simulink model "HornetXII_Challenge"  (R2026a)
settings: Solver=VariableStepAuto  StopTime=300  AbsTol=1e-3  EnableMultiTasking=on
InitFcn:
  | searchHalfSpan = 5;
  | 
  | rng('shuffle');
  | Environment.target.seed = randi(2^31 - 1);
  | 
  | % Use the saved seed to make this particular run reproducible if needed.
  | rng(Environment.target.seed, 'twister');
  | 
  | Environment.target.xy = (2*rand(2,1) - 1) * searchHalfSpan;
  | 
  | Environment.target.pos = [Environment.target.xy;
  |     Environment.seafloordepth - Environment.target.side/2];
values from neighbouring files (symbols this model uses):
  N = size(Vehicle.thrusterori, 2)    [VehicleParameters.m]
undefined symbols (not defined in the file or in its folder): B, pospoints, Spline, timepoints, Vehicle, X, Y, Z
libraries: sm_lib x554, nesl_utility x23, slpidlib x13, matrix_library x4, robotcorelib x2, fl_lib x1, simulink x1
(part 3 of 14)

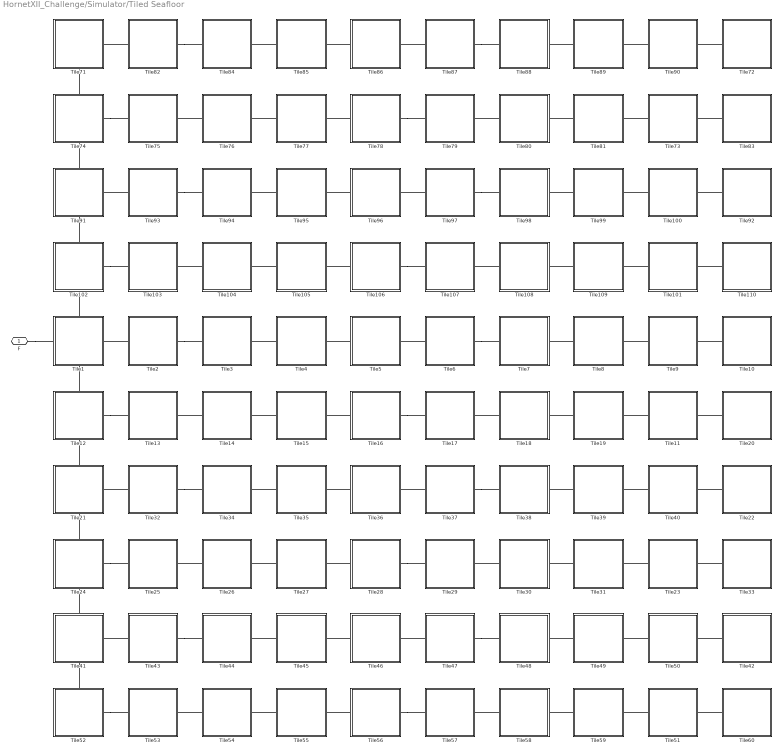
== system HornetXII_Challenge/Simulator/Tiled Seafloor ==
  Tile1 : Subsystem  mask(Square Tile){side=side, thickness=thick, color=color1, opacity=opacity}
      mask prompts: side "Side (m) :"; thickness "Thickness (m) :"; color "Color [RGB] :"; opacity "Opacity (0...1) :"
      mask help: This block creates a flat, single, square tile element. The square tile body is mass-less, so it will not have an effect on the dynamic simulation. This square tile element can be used as a graphic reference by itself, or as part of a composite graphic reference made of an array of interconnected tiles. The square tile is aligned with the XY plane, and the block provides frame connector ports to the middle points on each of the four sides of the body of the square - right (+X), left (-X), top (+Y) and bottom (-Y). All dimensions are in meters.
      settings: PortSchema="{\"entries\":[{\"content\":{\"sides\":[{\"content\":{\"connectorIds\":[\"LConn1\"]},\"type\":\"ConnectorPlacement.EquallySpacedRectSide\",\"uuid\":\"a971723f-ea37-4e9b-910b-501b94fb0ba2\"},{\"content\":{\"connectorIds\":[\"RConn1\"],\"side\":\"RIGHT\"},\"type\":\"ConnectorPlacement.EquallySpacedRectSide\",\"uuid\":\"e50175c1-005c-4b0b-bced-b882197eaab2\"},{\"content\":{\"connectorIds\":[\"LConn2\"],\"side\":\"TOP\"},\"type\":\"ConnectorPlacement.EquallySpacedRectSide\",\"uuid\":\"2a04a964-d53e-47ee-8c79-d53dd599bafe\"},{\"content\":{\"connectorIds\":[\"RConn2\"],\"side\":\"BOTTOM\"},\"type\":\"ConnectorPlacement.EquallySpacedRectSide\",\"uuid\":\"a0066dd6-a193-491c-afbe-bac00dfc3505\"}]},\"type\":\"ConnectorPlacement.EquallySpacedConnector\",\"uuid\":\"c80211c6-bb24-481b-97ca-2752015f3b18\"}],\"packageUris\":[\"http://schema.mathworks.com/mf0/Connector/19700101\"],\"version\":\"1.0\"}"
  Tile10 : Subsystem  mask(Square Tile){side=side, thickness=thick, color=color2, opacity=opacity}
      mask prompts: side "Side (m) :"; thickness "Thickness (m) :"; color "Color [RGB] :"; opacity "Opacity (0...1) :"
      mask help: This block creates a flat, single, square tile element. The square tile body is mass-less, so it will not have an effect on the dynamic simulation. This square tile element can be used as a graphic reference by itself, or as part of a composite graphic reference made of an array of interconnected tiles. The square tile is aligned with the XY plane, and the block provides frame connector ports to the middle points on each of the four sides of the body of the square - right (+X), left (-X), top (+Y) and bottom (-Y). All dimensions are in meters.
      settings: PortSchema="{\"entries\":[{\"content\":{\"sides\":[{\"content\":{\"connectorIds\":[\"LConn1\"]},\"type\":\"ConnectorPlacement.EquallySpacedRectSide\",\"uuid\":\"a971723f-ea37-4e9b-910b-501b94fb0ba2\"},{\"content\":{\"connectorIds\":[\"RConn1\"],\"side\":\"RIGHT\"},\"type\":\"ConnectorPlacement.EquallySpacedRectSide\",\"uuid\":\"e50175c1-005c-4b0b-bced-b882197eaab2\"},{\"content\":{\"connectorIds\":[\"LConn2\"],\"side\":\"TOP\"},\"type\":\"ConnectorPlacement.EquallySpacedRectSide\",\"uuid\":\"2a04a964-d53e-47ee-8c79-d53dd599bafe\"},{\"content\":{\"connectorIds\":[\"RConn2\"],\"side\":\"BOTTOM\"},\"type\":\"ConnectorPlacement.EquallySpacedRectSide\",\"uuid\":\"a0066dd6-a193-491c-afbe-bac00dfc3505\"}]},\"type\":\"ConnectorPlacement.EquallySpacedConnector\",\"uuid\":\"c80211c6-bb24-481b-97ca-2752015f3b18\"}],\"packageUris\":[\"http://schema.mathworks.com/mf0/Connector/19700101\"],\"version\":\"1.0\"}"
  Tile100 : Subsystem  mask(Square Tile){side=side, thickness=thick, color=color1, opacity=opacity}
      mask prompts: side "Side (m) :"; thickness "Thickness (m) :"; color "Color [RGB] :"; opacity "Opacity (0...1) :"
      mask help: This block creates a flat, single, square tile element. The square tile body is mass-less, so it will not have an effect on the dynamic simulation. This square tile element can be used as a graphic reference by itself, or as part of a composite graphic reference made of an array of interconnected tiles. The square tile is aligned with the XY plane, and the block provides frame connector ports to the middle points on each of the four sides of the body of the square - right (+X), left (-X), top (+Y) and bottom (-Y). All dimensions are in meters.
      settings: PortSchema="{\"entries\":[{\"content\":{\"sides\":[{\"content\":{\"connectorIds\":[\"LConn1\"]},\"type\":\"ConnectorPlacement.EquallySpacedRectSide\",\"uuid\":\"a971723f-ea37-4e9b-910b-501b94fb0ba2\"},{\"content\":{\"connectorIds\":[\"RConn1\"],\"side\":\"RIGHT\"},\"type\":\"ConnectorPlacement.EquallySpacedRectSide\",\"uuid\":\"e50175c1-005c-4b0b-bced-b882197eaab2\"},{\"content\":{\"connectorIds\":[\"LConn2\"],\"side\":\"TOP\"},\"type\":\"ConnectorPlacement.EquallySpacedRectSide\",\"uuid\":\"2a04a964-d53e-47ee-8c79-d53dd599bafe\"},{\"content\":{\"connectorIds\":[\"RConn2\"],\"side\":\"BOTTOM\"},\"type\":\"ConnectorPlacement.EquallySpacedRectSide\",\"uuid\":\"a0066dd6-a193-491c-afbe-bac00dfc3505\"}]},\"type\":\"ConnectorPlacement.EquallySpacedConnector\",\"uuid\":\"c80211c6-bb24-481b-97ca-2752015f3b18\"}],\"packageUris\":[\"http://schema.mathworks.com/mf0/Connector/19700101\"],\"version\":\"1.0\"}"
  Tile101 : Subsystem  mask(Square Tile){side=side, thickness=thick, color=color2, opacity=opacity}
      mask prompts: side "Side (m) :"; thickness "Thickness (m) :"; color "Color [RGB] :"; opacity "Opacity (0...1) :"
      mask help: This block creates a flat, single, square tile element. The square tile body is mass-less, so it will not have an effect on the dynamic simulation. This square tile element can be used as a graphic reference by itself, or as part of a composite graphic reference made of an array of interconnected tiles. The square tile is aligned with the XY plane, and the block provides frame connector ports to the middle points on each of the four sides of the body of the square - right (+X), left (-X), top (+Y) and bottom (-Y). All dimensions are in meters.
      settings: PortSchema="{\"entries\":[{\"content\":{\"sides\":[{\"content\":{\"connectorIds\":[\"LConn1\"]},\"type\":\"ConnectorPlacement.EquallySpacedRectSide\",\"uuid\":\"a971723f-ea37-4e9b-910b-501b94fb0ba2\"},{\"content\":{\"connectorIds\":[\"RConn1\"],\"side\":\"RIGHT\"},\"type\":\"ConnectorPlacement.EquallySpacedRectSide\",\"uuid\":\"e50175c1-005c-4b0b-bced-b882197eaab2\"},{\"content\":{\"connectorIds\":[\"LConn2\"],\"side\":\"TOP\"},\"type\":\"ConnectorPlacement.EquallySpacedRectSide\",\"uuid\":\"2a04a964-d53e-47ee-8c79-d53dd599bafe\"},{\"content\":{\"connectorIds\":[\"RConn2\"],\"side\":\"BOTTOM\"},\"type\":\"ConnectorPlacement.EquallySpacedRectSide\",\"uuid\":\"a0066dd6-a193-491c-afbe-bac00dfc3505\"}]},\"type\":\"ConnectorPlacement.EquallySpacedConnector\",\"uuid\":\"c80211c6-bb24-481b-97ca-2752015f3b18\"}],\"packageUris\":[\"http://schema.mathworks.com/mf0/Connector/19700101\"],\"version\":\"1.0\"}"
  Tile102 : Subsystem  mask(Square Tile){side=side, thickness=thick, color=color2, opacity=opacity}
      mask prompts: side "Side (m) :"; thickness "Thickness (m) :"; color "Color [RGB] :"; opacity "Opacity (0...1) :"
      mask help: This block creates a flat, single, square tile element. The square tile body is mass-less, so it will not have an effect on the dynamic simulation. This square tile element can be used as a graphic reference by itself, or as part of a composite graphic reference made of an array of interconnected tiles. The square tile is aligned with the XY plane, and the block provides frame connector ports to the middle points on each of the four sides of the body of the square - right (+X), left (-X), top (+Y) and bottom (-Y). All dimensions are in meters.
      settings: PortSchema="{\"entries\":[{\"content\":{\"sides\":[{\"content\":{\"connectorIds\":[\"LConn1\"]},\"type\":\"ConnectorPlacement.EquallySpacedRectSide\",\"uuid\":\"a971723f-ea37-4e9b-910b-501b94fb0ba2\"},{\"content\":{\"connectorIds\":[\"RConn1\"],\"side\":\"RIGHT\"},\"type\":\"ConnectorPlacement.EquallySpacedRectSide\",\"uuid\":\"e50175c1-005c-4b0b-bced-b882197eaab2\"},{\"content\":{\"connectorIds\":[\"LConn2\"],\"side\":\"TOP\"},\"type\":\"ConnectorPlacement.EquallySpacedRectSide\",\"uuid\":\"2a04a964-d53e-47ee-8c79-d53dd599bafe\"},{\"content\":{\"connectorIds\":[\"RConn2\"],\"side\":\"BOTTOM\"},\"type\":\"ConnectorPlacement.EquallySpacedRectSide\",\"uuid\":\"a0066dd6-a193-491c-afbe-bac00dfc3505\"}]},\"type\":\"ConnectorPlacement.EquallySpacedConnector\",\"uuid\":\"c80211c6-bb24-481b-97ca-2752015f3b18\"}],\"packageUris\":[\"http://schema.mathworks.com/mf0/Connector/19700101\"],\"version\":\"1.0\"}"
  Tile103 : Subsystem  mask(Square Tile){side=side, thickness=thick, color=color1, opacity=opacity}
      mask prompts: side "Side (m) :"; thickness "Thickness (m) :"; color "Color [RGB] :"; opacity "Opacity (0...1) :"
      mask help: This block creates a flat, single, square tile element. The square tile body is mass-less, so it will not have an effect on the dynamic simulation. This square tile element can be used as a graphic reference by itself, or as part of a composite graphic reference made of an array of interconnected tiles. The square tile is aligned with the XY plane, and the block provides frame connector ports to the middle points on each of the four sides of the body of the square - right (+X), left (-X), top (+Y) and bottom (-Y). All dimensions are in meters.
      settings: PortSchema="{\"entries\":[{\"content\":{\"sides\":[{\"content\":{\"connectorIds\":[\"LConn1\"]},\"type\":\"ConnectorPlacement.EquallySpacedRectSide\",\"uuid\":\"a971723f-ea37-4e9b-910b-501b94fb0ba2\"},{\"content\":{\"connectorIds\":[\"RConn1\"],\"side\":\"RIGHT\"},\"type\":\"ConnectorPlacement.EquallySpacedRectSide\",\"uuid\":\"e50175c1-005c-4b0b-bced-b882197eaab2\"},{\"content\":{\"connectorIds\":[\"LConn2\"],\"side\":\"TOP\"},\"type\":\"ConnectorPlacement.EquallySpacedRectSide\",\"uuid\":\"2a04a964-d53e-47ee-8c79-d53dd599bafe\"},{\"content\":{\"connectorIds\":[\"RConn2\"],\"side\":\"BOTTOM\"},\"type\":\"ConnectorPlacement.EquallySpacedRectSide\",\"uuid\":\"a0066dd6-a193-491c-afbe-bac00dfc3505\"}]},\"type\":\"ConnectorPlacement.EquallySpacedConnector\",\"uuid\":\"c80211c6-bb24-481b-97ca-2752015f3b18\"}],\"packageUris\":[\"http://schema.mathworks.com/mf0/Connector/19700101\"],\"version\":\"1.0\"}"
  Tile104 : Subsystem  mask(Square Tile){side=side, thickness=thick, color=color2, opacity=opacity}
      mask prompts: side "Side (m) :"; thickness "Thickness (m) :"; color "Color [RGB] :"; opacity "Opacity (0...1) :"
      mask help: This block creates a flat, single, square tile element. The square tile body is mass-less, so it will not have an effect on the dynamic simulation. This square tile element can be used as a graphic reference by itself, or as part of a composite graphic reference made of an array of interconnected tiles. The square tile is aligned with the XY plane, and the block provides frame connector ports to the middle points on each of the four sides of the body of the square - right (+X), left (-X), top (+Y) and bottom (-Y). All dimensions are in meters.
      settings: PortSchema="{\"entries\":[{\"content\":{\"sides\":[{\"content\":{\"connectorIds\":[\"LConn1\"]},\"type\":\"ConnectorPlacement.EquallySpacedRectSide\",\"uuid\":\"a971723f-ea37-4e9b-910b-501b94fb0ba2\"},{\"content\":{\"connectorIds\":[\"RConn1\"],\"side\":\"RIGHT\"},\"type\":\"ConnectorPlacement.EquallySpacedRectSide\",\"uuid\":\"e50175c1-005c-4b0b-bced-b882197eaab2\"},{\"content\":{\"connectorIds\":[\"LConn2\"],\"side\":\"TOP\"},\"type\":\"ConnectorPlacement.EquallySpacedRectSide\",\"uuid\":\"2a04a964-d53e-47ee-8c79-d53dd599bafe\"},{\"content\":{\"connectorIds\":[\"RConn2\"],\"side\":\"BOTTOM\"},\"type\":\"ConnectorPlacement.EquallySpacedRectSide\",\"uuid\":\"a0066dd6-a193-491c-afbe-bac00dfc3505\"}]},\"type\":\"ConnectorPlacement.EquallySpacedConnector\",\"uuid\":\"c80211c6-bb24-481b-97ca-2752015f3b18\"}],\"packageUris\":[\"http://schema.mathworks.com/mf0/Connector/19700101\"],\"version\":\"1.0\"}"
  Tile105 : Subsystem  mask(Square Tile){side=side, thickness=thick, color=color1, opacity=opacity}
      mask prompts: side "Side (m) :"; thickness "Thickness (m) :"; color "Color [RGB] :"; opacity "Opacity (0...1) :"
      mask help: This block creates a flat, single, square tile element. The square tile body is mass-less, so it will not have an effect on the dynamic simulation. This square tile element can be used as a graphic reference by itself, or as part of a composite graphic reference made of an array of interconnected tiles. The square tile is aligned with the XY plane, and the block provides frame connector ports to the middle points on each of the four sides of the body of the square - right (+X), left (-X), top (+Y) and bottom (-Y). All dimensions are in meters.
      settings: PortSchema="{\"entries\":[{\"content\":{\"sides\":[{\"content\":{\"connectorIds\":[\"LConn1\"]},\"type\":\"ConnectorPlacement.EquallySpacedRectSide\",\"uuid\":\"a971723f-ea37-4e9b-910b-501b94fb0ba2\"},{\"content\":{\"connectorIds\":[\"RConn1\"],\"side\":\"RIGHT\"},\"type\":\"ConnectorPlacement.EquallySpacedRectSide\",\"uuid\":\"e50175c1-005c-4b0b-bced-b882197eaab2\"},{\"content\":{\"connectorIds\":[\"LConn2\"],\"side\":\"TOP\"},\"type\":\"ConnectorPlacement.EquallySpacedRectSide\",\"uuid\":\"2a04a964-d53e-47ee-8c79-d53dd599bafe\"},{\"content\":{\"connectorIds\":[\"RConn2\"],\"side\":\"BOTTOM\"},\"type\":\"ConnectorPlacement.EquallySpacedRectSide\",\"uuid\":\"a0066dd6-a193-491c-afbe-bac00dfc3505\"}]},\"type\":\"ConnectorPlacement.EquallySpacedConnector\",\"uuid\":\"c80211c6-bb24-481b-97ca-2752015f3b18\"}],\"packageUris\":[\"http://schema.mathworks.com/mf0/Connector/19700101\"],\"version\":\"1.0\"}"
  Tile106 : Subsystem  mask(Square Tile){side=side, thickness=thick, color=color2, opacity=opacity}
      mask prompts: side "Side (m) :"; thickness "Thickness (m) :"; color "Color [RGB] :"; opacity "Opacity (0...1) :"
      mask help: This block creates a flat, single, square tile element. The square tile body is mass-less, so it will not have an effect on the dynamic simulation. This square tile element can be used as a graphic reference by itself, or as part of a composite graphic reference made of an array of interconnected tiles. The square tile is aligned with the XY plane, and the block provides frame connector ports to the middle points on each of the four sides of the body of the square - right (+X), left (-X), top (+Y) and bottom (-Y). All dimensions are in meters.
      settings: PortSchema="{\"entries\":[{\"content\":{\"sides\":[{\"content\":{\"connectorIds\":[\"LConn1\"]},\"type\":\"ConnectorPlacement.EquallySpacedRectSide\",\"uuid\":\"a971723f-ea37-4e9b-910b-501b94fb0ba2\"},{\"content\":{\"connectorIds\":[\"RConn1\"],\"side\":\"RIGHT\"},\"type\":\"ConnectorPlacement.EquallySpacedRectSide\",\"uuid\":\"e50175c1-005c-4b0b-bced-b882197eaab2\"},{\"content\":{\"connectorIds\":[\"LConn2\"],\"side\":\"TOP\"},\"type\":\"ConnectorPlacement.EquallySpacedRectSide\",\"uuid\":\"2a04a964-d53e-47ee-8c79-d53dd599bafe\"},{\"content\":{\"connectorIds\":[\"RConn2\"],\"side\":\"BOTTOM\"},\"type\":\"ConnectorPlacement.EquallySpacedRectSide\",\"uuid\":\"a0066dd6-a193-491c-afbe-bac00dfc3505\"}]},\"type\":\"ConnectorPlacement.EquallySpacedConnector\",\"uuid\":\"c80211c6-bb24-481b-97ca-2752015f3b18\"}],\"packageUris\":[\"http://schema.mathworks.com/mf0/Connector/19700101\"],\"version\":\"1.0\"}"
  Tile107 : Subsystem  mask(Square Tile){side=side, thickness=thick, color=color1, opacity=opacity}
      mask prompts: side "Side (m) :"; thickness "Thickness (m) :"; color "Color [RGB] :"; opacity "Opacity (0...1) :"
      mask help: This block creates a flat, single, square tile element. The square tile body is mass-less, so it will not have an effect on the dynamic simulation. This square tile element can be used as a graphic reference by itself, or as part of a composite graphic reference made of an array of interconnected tiles. The square tile is aligned with the XY plane, and the block provides frame connector ports to the middle points on each of the four sides of the body of the square - right (+X), left (-X), top (+Y) and bottom (-Y). All dimensions are in meters.
      settings: PortSchema="{\"entries\":[{\"content\":{\"sides\":[{\"content\":{\"connectorIds\":[\"LConn1\"]},\"type\":\"ConnectorPlacement.EquallySpacedRectSide\",\"uuid\":\"a971723f-ea37-4e9b-910b-501b94fb0ba2\"},{\"content\":{\"connectorIds\":[\"RConn1\"],\"side\":\"RIGHT\"},\"type\":\"ConnectorPlacement.EquallySpacedRectSide\",\"uuid\":\"e50175c1-005c-4b0b-bced-b882197eaab2\"},{\"content\":{\"connectorIds\":[\"LConn2\"],\"side\":\"TOP\"},\"type\":\"ConnectorPlacement.EquallySpacedRectSide\",\"uuid\":\"2a04a964-d53e-47ee-8c79-d53dd599bafe\"},{\"content\":{\"connectorIds\":[\"RConn2\"],\"side\":\"BOTTOM\"},\"type\":\"ConnectorPlacement.EquallySpacedRectSide\",\"uuid\":\"a0066dd6-a193-491c-afbe-bac00dfc3505\"}]},\"type\":\"ConnectorPlacement.EquallySpacedConnector\",\"uuid\":\"c80211c6-bb24-481b-97ca-2752015f3b18\"}],\"packageUris\":[\"http://schema.mathworks.com/mf0/Connector/19700101\"],\"version\":\"1.0\"}"
  Tile108 : Subsystem  mask(Square Tile){side=side, thickness=thick, color=color2, opacity=opacity}
      mask prompts: side "Side (m) :"; thickness "Thickness (m) :"; color "Color [RGB] :"; opacity "Opacity (0...1) :"
      mask help: This block creates a flat, single, square tile element. The square tile body is mass-less, so it will not have an effect on the dynamic simulation. This square tile element can be used as a graphic reference by itself, or as part of a composite graphic reference made of an array of interconnected tiles. The square tile is aligned with the XY plane, and the block provides frame connector ports to the middle points on each of the four sides of the body of the square - right (+X), left (-X), top (+Y) and bottom (-Y). All dimensions are in meters.
      settings: PortSchema="{\"entries\":[{\"content\":{\"sides\":[{\"content\":{\"connectorIds\":[\"LConn1\"]},\"type\":\"ConnectorPlacement.EquallySpacedRectSide\",\"uuid\":\"a971723f-ea37-4e9b-910b-501b94fb0ba2\"},{\"content\":{\"connectorIds\":[\"RConn1\"],\"side\":\"RIGHT\"},\"type\":\"ConnectorPlacement.EquallySpacedRectSide\",\"uuid\":\"e50175c1-005c-4b0b-bced-b882197eaab2\"},{\"content\":{\"connectorIds\":[\"LConn2\"],\"side\":\"TOP\"},\"type\":\"ConnectorPlacement.EquallySpacedRectSide\",\"uuid\":\"2a04a964-d53e-47ee-8c79-d53dd599bafe\"},{\"content\":{\"connectorIds\":[\"RConn2\"],\"side\":\"BOTTOM\"},\"type\":\"ConnectorPlacement.EquallySpacedRectSide\",\"uuid\":\"a0066dd6-a193-491c-afbe-bac00dfc3505\"}]},\"type\":\"ConnectorPlacement.EquallySpacedConnector\",\"uuid\":\"c80211c6-bb24-481b-97ca-2752015f3b18\"}],\"packageUris\":[\"http://schema.mathworks.com/mf0/Connector/19700101\"],\"version\":\"1.0\"}"
  Tile109 : Subsystem  mask(Square Tile){side=side, thickness=thick, color=color1, opacity=opacity}
      mask prompts: side "Side (m) :"; thickness "Thickness (m) :"; color "Color [RGB] :"; opacity "Opacity (0...1) :"
      mask help: This block creates a flat, single, square tile element. The square tile body is mass-less, so it will not have an effect on the dynamic simulation. This square tile element can be used as a graphic reference by itself, or as part of a composite graphic reference made of an array of interconnected tiles. The square tile is aligned with the XY plane, and the block provides frame connector ports to the middle points on each of the four sides of the body of the square - right (+X), left (-X), top (+Y) and bottom (-Y). All dimensions are in meters.
      settings: PortSchema="{\"entries\":[{\"content\":{\"sides\":[{\"content\":{\"connectorIds\":[\"LConn1\"]},\"type\":\"ConnectorPlacement.EquallySpacedRectSide\",\"uuid\":\"a971723f-ea37-4e9b-910b-501b94fb0ba2\"},{\"content\":{\"connectorIds\":[\"RConn1\"],\"side\":\"RIGHT\"},\"type\":\"ConnectorPlacement.EquallySpacedRectSide\",\"uuid\":\"e50175c1-005c-4b0b-bced-b882197eaab2\"},{\"content\":{\"connectorIds\":[\"LConn2\"],\"side\":\"TOP\"},\"type\":\"ConnectorPlacement.EquallySpacedRectSide\",\"uuid\":\"2a04a964-d53e-47ee-8c79-d53dd599bafe\"},{\"content\":{\"connectorIds\":[\"RConn2\"],\"side\":\"BOTTOM\"},\"type\":\"ConnectorPlacement.EquallySpacedRectSide\",\"uuid\":\"a0066dd6-a193-491c-afbe-bac00dfc3505\"}]},\"type\":\"ConnectorPlacement.EquallySpacedConnector\",\"uuid\":\"c80211c6-bb24-481b-97ca-2752015f3b18\"}],\"packageUris\":[\"http://schema.mathworks.com/mf0/Connector/19700101\"],\"version\":\"1.0\"}"
  Tile11 : Subsystem  mask(Square Tile){side=side, thickness=thick, color=color2, opacity=opacity}
      mask prompts: side "Side (m) :"; thickness "Thickness (m) :"; color "Color [RGB] :"; opacity "Opacity (0...1) :"
      mask help: This block creates a flat, single, square tile element. The square tile body is mass-less, so it will not have an effect on the dynamic simulation. This square tile element can be used as a graphic reference by itself, or as part of a composite graphic reference made of an array of interconnected tiles. The square tile is aligned with the XY plane, and the block provides frame connector ports to the middle points on each of the four sides of the body of the square - right (+X), left (-X), top (+Y) and bottom (-Y). All dimensions are in meters.
      settings: PortSchema="{\"entries\":[{\"content\":{\"sides\":[{\"content\":{\"connectorIds\":[\"LConn1\"]},\"type\":\"ConnectorPlacement.EquallySpacedRectSide\",\"uuid\":\"a971723f-ea37-4e9b-910b-501b94fb0ba2\"},{\"content\":{\"connectorIds\":[\"RConn1\"],\"side\":\"RIGHT\"},\"type\":\"ConnectorPlacement.EquallySpacedRectSide\",\"uuid\":\"e50175c1-005c-4b0b-bced-b882197eaab2\"},{\"content\":{\"connectorIds\":[\"LConn2\"],\"side\":\"TOP\"},\"type\":\"ConnectorPlacement.EquallySpacedRectSide\",\"uuid\":\"2a04a964-d53e-47ee-8c79-d53dd599bafe\"},{\"content\":{\"connectorIds\":[\"RConn2\"],\"side\":\"BOTTOM\"},\"type\":\"ConnectorPlacement.EquallySpacedRectSide\",\"uuid\":\"a0066dd6-a193-491c-afbe-bac00dfc3505\"}]},\"type\":\"ConnectorPlacement.EquallySpacedConnector\",\"uuid\":\"c80211c6-bb24-481b-97ca-2752015f3b18\"}],\"packageUris\":[\"http://schema.mathworks.com/mf0/Connector/19700101\"],\"version\":\"1.0\"}"
  Tile110 : Subsystem  mask(Square Tile){side=side, thickness=thick, color=color1, opacity=opacity}
      mask prompts: side "Side (m) :"; thickness "Thickness (m) :"; color "Color [RGB] :"; opacity "Opacity (0...1) :"
      mask help: This block creates a flat, single, square tile element. The square tile body is mass-less, so it will not have an effect on the dynamic simulation. This square tile element can be used as a graphic reference by itself, or as part of a composite graphic reference made of an array of interconnected tiles. The square tile is aligned with the XY plane, and the block provides frame connector ports to the middle points on each of the four sides of the body of the square - right (+X), left (-X), top (+Y) and bottom (-Y). All dimensions are in meters.
      settings: PortSchema="{\"entries\":[{\"content\":{\"sides\":[{\"content\":{\"connectorIds\":[\"LConn1\"]},\"type\":\"ConnectorPlacement.EquallySpacedRectSide\",\"uuid\":\"a971723f-ea37-4e9b-910b-501b94fb0ba2\"},{\"content\":{\"connectorIds\":[\"RConn1\"],\"side\":\"RIGHT\"},\"type\":\"ConnectorPlacement.EquallySpacedRectSide\",\"uuid\":\"e50175c1-005c-4b0b-bced-b882197eaab2\"},{\"content\":{\"connectorIds\":[\"LConn2\"],\"side\":\"TOP\"},\"type\":\"ConnectorPlacement.EquallySpacedRectSide\",\"uuid\":\"2a04a964-d53e-47ee-8c79-d53dd599bafe\"},{\"content\":{\"connectorIds\":[\"RConn2\"],\"side\":\"BOTTOM\"},\"type\":\"ConnectorPlacement.EquallySpacedRectSide\",\"uuid\":\"a0066dd6-a193-491c-afbe-bac00dfc3505\"}]},\"type\":\"ConnectorPlacement.EquallySpacedConnector\",\"uuid\":\"c80211c6-bb24-481b-97ca-2752015f3b18\"}],\"packageUris\":[\"http://schema.mathworks.com/mf0/Connector/19700101\"],\"version\":\"1.0\"}"
  Tile12 : Subsystem  mask(Square Tile){side=side, thickness=thick, color=color2, opacity=opacity}
      mask prompts: side "Side (m) :"; thickness "Thickness (m) :"; color "Color [RGB] :"; opacity "Opacity (0...1) :"
      mask help: This block creates a flat, single, square tile element. The square tile body is mass-less, so it will not have an effect on the dynamic simulation. This square tile element can be used as a graphic reference by itself, or as part of a composite graphic reference made of an array of interconnected tiles. The square tile is aligned with the XY plane, and the block provides frame connector ports to the middle points on each of the four sides of the body of the square - right (+X), left (-X), top (+Y) and bottom (-Y). All dimensions are in meters.
      settings: PortSchema="{\"entries\":[{\"content\":{\"sides\":[{\"content\":{\"connectorIds\":[\"LConn1\"]},\"type\":\"ConnectorPlacement.EquallySpacedRectSide\",\"uuid\":\"a971723f-ea37-4e9b-910b-501b94fb0ba2\"},{\"content\":{\"connectorIds\":[\"RConn1\"],\"side\":\"RIGHT\"},\"type\":\"ConnectorPlacement.EquallySpacedRectSide\",\"uuid\":\"e50175c1-005c-4b0b-bced-b882197eaab2\"},{\"content\":{\"connectorIds\":[\"LConn2\"],\"side\":\"TOP\"},\"type\":\"ConnectorPlacement.EquallySpacedRectSide\",\"uuid\":\"2a04a964-d53e-47ee-8c79-d53dd599bafe\"},{\"content\":{\"connectorIds\":[\"RConn2\"],\"side\":\"BOTTOM\"},\"type\":\"ConnectorPlacement.EquallySpacedRectSide\",\"uuid\":\"a0066dd6-a193-491c-afbe-bac00dfc3505\"}]},\"type\":\"ConnectorPlacement.EquallySpacedConnector\",\"uuid\":\"c80211c6-bb24-481b-97ca-2752015f3b18\"}],\"packageUris\":[\"http://schema.mathworks.com/mf0/Connector/19700101\"],\"version\":\"1.0\"}"
  Tile13 : Subsystem  mask(Square Tile){side=side, thickness=thick, color=color1, opacity=opacity}
      mask prompts: side "Side (m) :"; thickness "Thickness (m) :"; color "Color [RGB] :"; opacity "Opacity (0...1) :"
      mask help: This block creates a flat, single, square tile element. The square tile body is mass-less, so it will not have an effect on the dynamic simulation. This square tile element can be used as a graphic reference by itself, or as part of a composite graphic reference made of an array of interconnected tiles. The square tile is aligned with the XY plane, and the block provides frame connector ports to the middle points on each of the four sides of the body of the square - right (+X), left (-X), top (+Y) and bottom (-Y). All dimensions are in meters.
      settings: PortSchema="{\"entries\":[{\"content\":{\"sides\":[{\"content\":{\"connectorIds\":[\"LConn1\"]},\"type\":\"ConnectorPlacement.EquallySpacedRectSide\",\"uuid\":\"a971723f-ea37-4e9b-910b-501b94fb0ba2\"},{\"content\":{\"connectorIds\":[\"RConn1\"],\"side\":\"RIGHT\"},\"type\":\"ConnectorPlacement.EquallySpacedRectSide\",\"uuid\":\"e50175c1-005c-4b0b-bced-b882197eaab2\"},{\"content\":{\"connectorIds\":[\"LConn2\"],\"side\":\"TOP\"},\"type\":\"ConnectorPlacement.EquallySpacedRectSide\",\"uuid\":\"2a04a964-d53e-47ee-8c79-d53dd599bafe\"},{\"content\":{\"connectorIds\":[\"RConn2\"],\"side\":\"BOTTOM\"},\"type\":\"ConnectorPlacement.EquallySpacedRectSide\",\"uuid\":\"a0066dd6-a193-491c-afbe-bac00dfc3505\"}]},\"type\":\"ConnectorPlacement.EquallySpacedConnector\",\"uuid\":\"c80211c6-bb24-481b-97ca-2752015f3b18\"}],\"packageUris\":[\"http://schema.mathworks.com/mf0/Connector/19700101\"],\"version\":\"1.0\"}"
  Tile14 : Subsystem  mask(Square Tile){side=side, thickness=thick, color=color2, opacity=opacity}
      mask prompts: side "Side (m) :"; thickness "Thickness (m) :"; color "Color [RGB] :"; opacity "Opacity (0...1) :"
      mask help: This block creates a flat, single, square tile element. The square tile body is mass-less, so it will not have an effect on the dynamic simulation. This square tile element can be used as a graphic reference by itself, or as part of a composite graphic reference made of an array of interconnected tiles. The square tile is aligned with the XY plane, and the block provides frame connector ports to the middle points on each of the four sides of the body of the square - right (+X), left (-X), top (+Y) and bottom (-Y). All dimensions are in meters.
      settings: PortSchema="{\"entries\":[{\"content\":{\"sides\":[{\"content\":{\"connectorIds\":[\"LConn1\"]},\"type\":\"ConnectorPlacement.EquallySpacedRectSide\",\"uuid\":\"a971723f-ea37-4e9b-910b-501b94fb0ba2\"},{\"content\":{\"connectorIds\":[\"RConn1\"],\"side\":\"RIGHT\"},\"type\":\"ConnectorPlacement.EquallySpacedRectSide\",\"uuid\":\"e50175c1-005c-4b0b-bced-b882197eaab2\"},{\"content\":{\"connectorIds\":[\"LConn2\"],\"side\":\"TOP\"},\"type\":\"ConnectorPlacement.EquallySpacedRectSide\",\"uuid\":\"2a04a964-d53e-47ee-8c79-d53dd599bafe\"},{\"content\":{\"connectorIds\":[\"RConn2\"],\"side\":\"BOTTOM\"},\"type\":\"ConnectorPlacement.EquallySpacedRectSide\",\"uuid\":\"a0066dd6-a193-491c-afbe-bac00dfc3505\"}]},\"type\":\"ConnectorPlacement.EquallySpacedConnector\",\"uuid\":\"c80211c6-bb24-481b-97ca-2752015f3b18\"}],\"packageUris\":[\"http://schema.mathworks.com/mf0/Connector/19700101\"],\"version\":\"1.0\"}"
  Tile15 : Subsystem  mask(Square Tile){side=side, thickness=thick, color=color1, opacity=opacity}
      mask prompts: side "Side (m) :"; thickness "Thickness (m) :"; color "Color [RGB] :"; opacity "Opacity (0...1) :"
      mask help: This block creates a flat, single, square tile element. The square tile body is mass-less, so it will not have an effect on the dynamic simulation. This square tile element can be used as a graphic reference by itself, or as part of a composite graphic reference made of an array of interconnected tiles. The square tile is aligned with the XY plane, and the block provides frame connector ports to the middle points on each of the four sides of the body of the square - right (+X), left (-X), top (+Y) and bottom (-Y). All dimensions are in meters.
      settings: PortSchema="{\"entries\":[{\"content\":{\"sides\":[{\"content\":{\"connectorIds\":[\"LConn1\"]},\"type\":\"ConnectorPlacement.EquallySpacedRectSide\",\"uuid\":\"a971723f-ea37-4e9b-910b-501b94fb0ba2\"},{\"content\":{\"connectorIds\":[\"RConn1\"],\"side\":\"RIGHT\"},\"type\":\"ConnectorPlacement.EquallySpacedRectSide\",\"uuid\":\"e50175c1-005c-4b0b-bced-b882197eaab2\"},{\"content\":{\"connectorIds\":[\"LConn2\"],\"side\":\"TOP\"},\"type\":\"ConnectorPlacement.EquallySpacedRectSide\",\"uuid\":\"2a04a964-d53e-47ee-8c79-d53dd599bafe\"},{\"content\":{\"connectorIds\":[\"RConn2\"],\"side\":\"BOTTOM\"},\"type\":\"ConnectorPlacement.EquallySpacedRectSide\",\"uuid\":\"a0066dd6-a193-491c-afbe-bac00dfc3505\"}]},\"type\":\"ConnectorPlacement.EquallySpacedConnector\",\"uuid\":\"c80211c6-bb24-481b-97ca-2752015f3b18\"}],\"packageUris\":[\"http://schema.mathworks.com/mf0/Connector/19700101\"],\"version\":\"1.0\"}"
  Tile16 : Subsystem  mask(Square Tile){side=side, thickness=thick, color=color2, opacity=opacity}
      mask prompts: side "Side (m) :"; thickness "Thickness (m) :"; color "Color [RGB] :"; opacity "Opacity (0...1) :"
      mask help: This block creates a flat, single, square tile element. The square tile body is mass-less, so it will not have an effect on the dynamic simulation. This square tile element can be used as a graphic reference by itself, or as part of a composite graphic reference made of an array of interconnected tiles. The square tile is aligned with the XY plane, and the block provides frame connector ports to the middle points on each of the four sides of the body of the square - right (+X), left (-X), top (+Y) and bottom (-Y). All dimensions are in meters.
      settings: PortSchema="{\"entries\":[{\"content\":{\"sides\":[{\"content\":{\"connectorIds\":[\"LConn1\"]},\"type\":\"ConnectorPlacement.EquallySpacedRectSide\",\"uuid\":\"a971723f-ea37-4e9b-910b-501b94fb0ba2\"},{\"content\":{\"connectorIds\":[\"RConn1\"],\"side\":\"RIGHT\"},\"type\":\"ConnectorPlacement.EquallySpacedRectSide\",\"uuid\":\"e50175c1-005c-4b0b-bced-b882197eaab2\"},{\"content\":{\"connectorIds\":[\"LConn2\"],\"side\":\"TOP\"},\"type\":\"ConnectorPlacement.EquallySpacedRectSide\",\"uuid\":\"2a04a964-d53e-47ee-8c79-d53dd599bafe\"},{\"content\":{\"connectorIds\":[\"RConn2\"],\"side\":\"BOTTOM\"},\"type\":\"ConnectorPlacement.EquallySpacedRectSide\",\"uuid\":\"a0066dd6-a193-491c-afbe-bac00dfc3505\"}]},\"type\":\"ConnectorPlacement.EquallySpacedConnector\",\"uuid\":\"c80211c6-bb24-481b-97ca-2752015f3b18\"}],\"packageUris\":[\"http://schema.mathworks.com/mf0/Connector/19700101\"],\"version\":\"1.0\"}"
  Tile17 : Subsystem  mask(Square Tile){side=side, thickness=thick, color=color1, opacity=opacity}
      mask prompts: side "Side (m) :"; thickness "Thickness (m) :"; color "Color [RGB] :"; opacity "Opacity (0...1) :"
      mask help: This block creates a flat, single, square tile element. The square tile body is mass-less, so it will not have an effect on the dynamic simulation. This square tile element can be used as a graphic reference by itself, or as part of a composite graphic reference made of an array of interconnected tiles. The square tile is aligned with the XY plane, and the block provides frame connector ports to the middle points on each of the four sides of the body of the square - right (+X), left (-X), top (+Y) and bottom (-Y). All dimensions are in meters.
      settings: PortSchema="{\"entries\":[{\"content\":{\"sides\":[{\"content\":{\"connectorIds\":[\"LConn1\"]},\"type\":\"ConnectorPlacement.EquallySpacedRectSide\",\"uuid\":\"a971723f-ea37-4e9b-910b-501b94fb0ba2\"},{\"content\":{\"connectorIds\":[\"RConn1\"],\"side\":\"RIGHT\"},\"type\":\"ConnectorPlacement.EquallySpacedRectSide\",\"uuid\":\"e50175c1-005c-4b0b-bced-b882197eaab2\"},{\"content\":{\"connectorIds\":[\"LConn2\"],\"side\":\"TOP\"},\"type\":\"ConnectorPlacement.EquallySpacedRectSide\",\"uuid\":\"2a04a964-d53e-47ee-8c79-d53dd599bafe\"},{\"content\":{\"connectorIds\":[\"RConn2\"],\"side\":\"BOTTOM\"},\"type\":\"ConnectorPlacement.EquallySpacedRectSide\",\"uuid\":\"a0066dd6-a193-491c-afbe-bac00dfc3505\"}]},\"type\":\"ConnectorPlacement.EquallySpacedConnector\",\"uuid\":\"c80211c6-bb24-481b-97ca-2752015f3b18\"}],\"packageUris\":[\"http://schema.mathworks.com/mf0/Connector/19700101\"],\"version\":\"1.0\"}"
  Tile18 : Subsystem  mask(Square Tile){side=side, thickness=thick, color=color2, opacity=opacity}
      mask prompts: side "Side (m) :"; thickness "Thickness (m) :"; color "Color [RGB] :"; opacity "Opacity (0...1) :"
      mask help: This block creates a flat, single, square tile element. The square tile body is mass-less, so it will not have an effect on the dynamic simulation. This square tile element can be used as a graphic reference by itself, or as part of a composite graphic reference made of an array of interconnected tiles. The square tile is aligned with the XY plane, and the block provides frame connector ports to the middle points on each of the four sides of the body of the square - right (+X), left (-X), top (+Y) and bottom (-Y). All dimensions are in meters.
      settings: PortSchema="{\"entries\":[{\"content\":{\"sides\":[{\"content\":{\"connectorIds\":[\"LConn1\"]},\"type\":\"ConnectorPlacement.EquallySpacedRectSide\",\"uuid\":\"a971723f-ea37-4e9b-910b-501b94fb0ba2\"},{\"content\":{\"connectorIds\":[\"RConn1\"],\"side\":\"RIGHT\"},\"type\":\"ConnectorPlacement.EquallySpacedRectSide\",\"uuid\":\"e50175c1-005c-4b0b-bced-b882197eaab2\"},{\"content\":{\"connectorIds\":[\"LConn2\"],\"side\":\"TOP\"},\"type\":\"ConnectorPlacement.EquallySpacedRectSide\",\"uuid\":\"2a04a964-d53e-47ee-8c79-d53dd599bafe\"},{\"content\":{\"connectorIds\":[\"RConn2\"],\"side\":\"BOTTOM\"},\"type\":\"ConnectorPlacement.EquallySpacedRectSide\",\"uuid\":\"a0066dd6-a193-491c-afbe-bac00dfc3505\"}]},\"type\":\"ConnectorPlacement.EquallySpacedConnector\",\"uuid\":\"c80211c6-bb24-481b-97ca-2752015f3b18\"}],\"packageUris\":[\"http://schema.mathworks.com/mf0/Connector/19700101\"],\"version\":\"1.0\"}"
  Tile19 : Subsystem  mask(Square Tile){side=side, thickness=thick, color=color1, opacity=opacity}
      mask prompts: side "Side (m) :"; thickness "Thickness (m) :"; color "Color [RGB] :"; opacity "Opacity (0...1) :"
      mask help: This block creates a flat, single, square tile element. The square tile body is mass-less, so it will not have an effect on the dynamic simulation. This square tile element can be used as a graphic reference by itself, or as part of a composite graphic reference made of an array of interconnected tiles. The square tile is aligned with the XY plane, and the block provides frame connector ports to the middle points on each of the four sides of the body of the square - right (+X), left (-X), top (+Y) and bottom (-Y). All dimensions are in meters.
      settings: PortSchema="{\"entries\":[{\"content\":{\"sides\":[{\"content\":{\"connectorIds\":[\"LConn1\"]},\"type\":\"ConnectorPlacement.EquallySpacedRectSide\",\"uuid\":\"a971723f-ea37-4e9b-910b-501b94fb0ba2\"},{\"content\":{\"connectorIds\":[\"RConn1\"],\"side\":\"RIGHT\"},\"type\":\"ConnectorPlacement.EquallySpacedRectSide\",\"uuid\":\"e50175c1-005c-4b0b-bced-b882197eaab2\"},{\"content\":{\"connectorIds\":[\"LConn2\"],\"side\":\"TOP\"},\"type\":\"ConnectorPlacement.EquallySpacedRectSide\",\"uuid\":\"2a04a964-d53e-47ee-8c79-d53dd599bafe\"},{\"content\":{\"connectorIds\":[\"RConn2\"],\"side\":\"BOTTOM\"},\"type\":\"ConnectorPlacement.EquallySpacedRectSide\",\"uuid\":\"a0066dd6-a193-491c-afbe-bac00dfc3505\"}]},\"type\":\"ConnectorPlacement.EquallySpacedConnector\",\"uuid\":\"c80211c6-bb24-481b-97ca-2752015f3b18\"}],\"packageUris\":[\"http://schema.mathworks.com/mf0/Connector/19700101\"],\"version\":\"1.0\"}"
  Tile2 : Subsystem  mask(Square Tile){side=side, thickness=thick, color=color2, opacity=opacity}
      mask prompts: side "Side (m) :"; thickness "Thickness (m) :"; color "Color [RGB] :"; opacity "Opacity (0...1) :"
      mask help: This block creates a flat, single, square tile element. The square tile body is mass-less, so it will not have an effect on the dynamic simulation. This square tile element can be used as a graphic reference by itself, or as part of a composite graphic reference made of an array of interconnected tiles. The square tile is aligned with the XY plane, and the block provides frame connector ports to the middle points on each of the four sides of the body of the square - right (+X), left (-X), top (+Y) and bottom (-Y). All dimensions are in meters.
      settings: PortSchema="{\"entries\":[{\"content\":{\"sides\":[{\"content\":{\"connectorIds\":[\"LConn1\"]},\"type\":\"ConnectorPlacement.EquallySpacedRectSide\",\"uuid\":\"a971723f-ea37-4e9b-910b-501b94fb0ba2\"},{\"content\":{\"connectorIds\":[\"RConn1\"],\"side\":\"RIGHT\"},\"type\":\"ConnectorPlacement.EquallySpacedRectSide\",\"uuid\":\"e50175c1-005c-4b0b-bced-b882197eaab2\"},{\"content\":{\"connectorIds\":[\"LConn2\"],\"side\":\"TOP\"},\"type\":\"ConnectorPlacement.EquallySpacedRectSide\",\"uuid\":\"2a04a964-d53e-47ee-8c79-d53dd599bafe\"},{\"content\":{\"connectorIds\":[\"RConn2\"],\"side\":\"BOTTOM\"},\"type\":\"ConnectorPlacement.EquallySpacedRectSide\",\"uuid\":\"a0066dd6-a193-491c-afbe-bac00dfc3505\"}]},\"type\":\"ConnectorPlacement.EquallySpacedConnector\",\"uuid\":\"c80211c6-bb24-481b-97ca-2752015f3b18\"}],\"packageUris\":[\"http://schema.mathworks.com/mf0/Connector/19700101\"],\"version\":\"1.0\"}"
  Tile20 : Subsystem  mask(Square Tile){side=side, thickness=thick, color=color1, opacity=opacity}
      mask prompts: side "Side (m) :"; thickness "Thickness (m) :"; color "Color [RGB] :"; opacity "Opacity (0...1) :"
      mask help: This block creates a flat, single, square tile element. The square tile body is mass-less, so it will not have an effect on the dynamic simulation. This square tile element can be used as a graphic reference by itself, or as part of a composite graphic reference made of an array of interconnected tiles. The square tile is aligned with the XY plane, and the block provides frame connector ports to the middle points on each of the four sides of the body of the square - right (+X), left (-X), top (+Y) and bottom (-Y). All dimensions are in meters.
      settings: PortSchema="{\"entries\":[{\"content\":{\"sides\":[{\"content\":{\"connectorIds\":[\"LConn1\"]},\"type\":\"ConnectorPlacement.EquallySpacedRectSide\",\"uuid\":\"a971723f-ea37-4e9b-910b-501b94fb0ba2\"},{\"content\":{\"connectorIds\":[\"RConn1\"],\"side\":\"RIGHT\"},\"type\":\"ConnectorPlacement.EquallySpacedRectSide\",\"uuid\":\"e50175c1-005c-4b0b-bced-b882197eaab2\"},{\"content\":{\"connectorIds\":[\"LConn2\"],\"side\":\"TOP\"},\"type\":\"ConnectorPlacement.EquallySpacedRectSide\",\"uuid\":\"2a04a964-d53e-47ee-8c79-d53dd599bafe\"},{\"content\":{\"connectorIds\":[\"RConn2\"],\"side\":\"BOTTOM\"},\"type\":\"ConnectorPlacement.EquallySpacedRectSide\",\"uuid\":\"a0066dd6-a193-491c-afbe-bac00dfc3505\"}]},\"type\":\"ConnectorPlacement.EquallySpacedConnector\",\"uuid\":\"c80211c6-bb24-481b-97ca-2752015f3b18\"}],\"packageUris\":[\"http://schema.mathworks.com/mf0/Connector/19700101\"],\"version\":\"1.0\"}"
  Tile21 : Subsystem  mask(Square Tile){side=side, thickness=thick, color=color1, opacity=opacity}
      mask prompts: side "Side (m) :"; thickness "Thickness (m) :"; color "Color [RGB] :"; opacity "Opacity (0...1) :"
      mask help: This block creates a flat, single, square tile element. The square tile body is mass-less, so it will not have an effect on the dynamic simulation. This square tile element can be used as a graphic reference by itself, or as part of a composite graphic reference made of an array of interconnected tiles. The square tile is aligned with the XY plane, and the block provides frame connector ports to the middle points on each of the four sides of the body of the square - right (+X), left (-X), top (+Y) and bottom (-Y). All dimensions are in meters.
      settings: PortSchema="{\"entries\":[{\"content\":{\"sides\":[{\"content\":{\"connectorIds\":[\"LConn1\"]},\"type\":\"ConnectorPlacement.EquallySpacedRectSide\",\"uuid\":\"a971723f-ea37-4e9b-910b-501b94fb0ba2\"},{\"content\":{\"connectorIds\":[\"RConn1\"],\"side\":\"RIGHT\"},\"type\":\"ConnectorPlacement.EquallySpacedRectSide\",\"uuid\":\"e50175c1-005c-4b0b-bced-b882197eaab2\"},{\"content\":{\"connectorIds\":[\"LConn2\"],\"side\":\"TOP\"},\"type\":\"ConnectorPlacement.EquallySpacedRectSide\",\"uuid\":\"2a04a964-d53e-47ee-8c79-d53dd599bafe\"},{\"content\":{\"connectorIds\":[\"RConn2\"],\"side\":\"BOTTOM\"},\"type\":\"ConnectorPlacement.EquallySpacedRectSide\",\"uuid\":\"a0066dd6-a193-491c-afbe-bac00dfc3505\"}]},\"type\":\"ConnectorPlacement.EquallySpacedConnector\",\"uuid\":\"c80211c6-bb24-481b-97ca-2752015f3b18\"}],\"packageUris\":[\"http://schema.mathworks.com/mf0/Connector/19700101\"],\"version\":\"1.0\"}"
  Tile22 : Subsystem  mask(Square Tile){side=side, thickness=thick, color=color2, opacity=opacity}
      mask prompts: side "Side (m) :"; thickness "Thickness (m) :"; color "Color [RGB] :"; opacity "Opacity (0...1) :"
      mask help: This block creates a flat, single, square tile element. The square tile body is mass-less, so it will not have an effect on the dynamic simulation. This square tile element can be used as a graphic reference by itself, or as part of a composite graphic reference made of an array of interconnected tiles. The square tile is aligned with the XY plane, and the block provides frame connector ports to the middle points on each of the four sides of the body of the square - right (+X), left (-X), top (+Y) and bottom (-Y). All dimensions are in meters.
      settings: PortSchema="{\"entries\":[{\"content\":{\"sides\":[{\"content\":{\"connectorIds\":[\"LConn1\"]},\"type\":\"ConnectorPlacement.EquallySpacedRectSide\",\"uuid\":\"a971723f-ea37-4e9b-910b-501b94fb0ba2\"},{\"content\":{\"connectorIds\":[\"RConn1\"],\"side\":\"RIGHT\"},\"type\":\"ConnectorPlacement.EquallySpacedRectSide\",\"uuid\":\"e50175c1-005c-4b0b-bced-b882197eaab2\"},{\"content\":{\"connectorIds\":[\"LConn2\"],\"side\":\"TOP\"},\"type\":\"ConnectorPlacement.EquallySpacedRectSide\",\"uuid\":\"2a04a964-d53e-47ee-8c79-d53dd599bafe\"},{\"content\":{\"connectorIds\":[\"RConn2\"],\"side\":\"BOTTOM\"},\"type\":\"ConnectorPlacement.EquallySpacedRectSide\",\"uuid\":\"a0066dd6-a193-491c-afbe-bac00dfc3505\"}]},\"type\":\"ConnectorPlacement.EquallySpacedConnector\",\"uuid\":\"c80211c6-bb24-481b-97ca-2752015f3b18\"}],\"packageUris\":[\"http://schema.mathworks.com/mf0/Connector/19700101\"],\"version\":\"1.0\"}"
  Tile23 : Subsystem  mask(Square Tile){side=side, thickness=thick, color=color2, opacity=opacity}
      mask prompts: side "Side (m) :"; thickness "Thickness (m) :"; color "Color [RGB] :"; opacity "Opacity (0...1) :"
      mask help: This block creates a flat, single, square tile element. The square tile body is mass-less, so it will not have an effect on the dynamic simulation. This square tile element can be used as a graphic reference by itself, or as part of a composite graphic reference made of an array of interconnected tiles. The square tile is aligned with the XY plane, and the block provides frame connector ports to the middle points on each of the four sides of the body of the square - right (+X), left (-X), top (+Y) and bottom (-Y). All dimensions are in meters.
      settings: PortSchema="{\"entries\":[{\"content\":{\"sides\":[{\"content\":{\"connectorIds\":[\"LConn1\"]},\"type\":\"ConnectorPlacement.EquallySpacedRectSide\",\"uuid\":\"a971723f-ea37-4e9b-910b-501b94fb0ba2\"},{\"content\":{\"connectorIds\":[\"RConn1\"],\"side\":\"RIGHT\"},\"type\":\"ConnectorPlacement.EquallySpacedRectSide\",\"uuid\":\"e50175c1-005c-4b0b-bced-b882197eaab2\"},{\"content\":{\"connectorIds\":[\"LConn2\"],\"side\":\"TOP\"},\"type\":\"ConnectorPlacement.EquallySpacedRectSide\",\"uuid\":\"2a04a964-d53e-47ee-8c79-d53dd599bafe\"},{\"content\":{\"connectorIds\":[\"RConn2\"],\"side\":\"BOTTOM\"},\"type\":\"ConnectorPlacement.EquallySpacedRectSide\",\"uuid\":\"a0066dd6-a193-491c-afbe-bac00dfc3505\"}]},\"type\":\"ConnectorPlacement.EquallySpacedConnector\",\"uuid\":\"c80211c6-bb24-481b-97ca-2752015f3b18\"}],\"packageUris\":[\"http://schema.mathworks.com/mf0/Connector/19700101\"],\"version\":\"1.0\"}"
  Tile24 : Subsystem  mask(Square Tile){side=side, thickness=thick, color=color2, opacity=opacity}
      mask prompts: side "Side (m) :"; thickness "Thickness (m) :"; color "Color [RGB] :"; opacity "Opacity (0...1) :"
      mask help: This block creates a flat, single, square tile element. The square tile body is mass-less, so it will not have an effect on the dynamic simulation. This square tile element can be used as a graphic reference by itself, or as part of a composite graphic reference made of an array of interconnected tiles. The square tile is aligned with the XY plane, and the block provides frame connector ports to the middle points on each of the four sides of the body of the square - right (+X), left (-X), top (+Y) and bottom (-Y). All dimensions are in meters.
      settings: PortSchema="{\"entries\":[{\"content\":{\"sides\":[{\"content\":{\"connectorIds\":[\"LConn1\"]},\"type\":\"ConnectorPlacement.EquallySpacedRectSide\",\"uuid\":\"a971723f-ea37-4e9b-910b-501b94fb0ba2\"},{\"content\":{\"connectorIds\":[\"RConn1\"],\"side\":\"RIGHT\"},\"type\":\"ConnectorPlacement.EquallySpacedRectSide\",\"uuid\":\"e50175c1-005c-4b0b-bced-b882197eaab2\"},{\"content\":{\"connectorIds\":[\"LConn2\"],\"side\":\"TOP\"},\"type\":\"ConnectorPlacement.EquallySpacedRectSide\",\"uuid\":\"2a04a964-d53e-47ee-8c79-d53dd599bafe\"},{\"content\":{\"connectorIds\":[\"RConn2\"],\"side\":\"BOTTOM\"},\"type\":\"ConnectorPlacement.EquallySpacedRectSide\",\"uuid\":\"a0066dd6-a193-491c-afbe-bac00dfc3505\"}]},\"type\":\"ConnectorPlacement.EquallySpacedConnector\",\"uuid\":\"c80211c6-bb24-481b-97ca-2752015f3b18\"}],\"packageUris\":[\"http://schema.mathworks.com/mf0/Connector/19700101\"],\"version\":\"1.0\"}"
  Tile25 : Subsystem  mask(Square Tile){side=side, thickness=thick, color=color1, opacity=opacity}
      mask prompts: side "Side (m) :"; thickness "Thickness (m) :"; color "Color [RGB] :"; opacity "Opacity (0...1) :"
      mask help: This block creates a flat, single, square tile element. The square tile body is mass-less, so it will not have an effect on the dynamic simulation. This square tile element can be used as a graphic reference by itself, or as part of a composite graphic reference made of an array of interconnected tiles. The square tile is aligned with the XY plane, and the block provides frame connector ports to the middle points on each of the four sides of the body of the square - right (+X), left (-X), top (+Y) and bottom (-Y). All dimensions are in meters.
      settings: PortSchema="{\"entries\":[{\"content\":{\"sides\":[{\"content\":{\"connectorIds\":[\"LConn1\"]},\"type\":\"ConnectorPlacement.EquallySpacedRectSide\",\"uuid\":\"a971723f-ea37-4e9b-910b-501b94fb0ba2\"},{\"content\":{\"connectorIds\":[\"RConn1\"],\"side\":\"RIGHT\"},\"type\":\"ConnectorPlacement.EquallySpacedRectSide\",\"uuid\":\"e50175c1-005c-4b0b-bced-b882197eaab2\"},{\"content\":{\"connectorIds\":[\"LConn2\"],\"side\":\"TOP\"},\"type\":\"ConnectorPlacement.EquallySpacedRectSide\",\"uuid\":\"2a04a964-d53e-47ee-8c79-d53dd599bafe\"},{\"content\":{\"connectorIds\":[\"RConn2\"],\"side\":\"BOTTOM\"},\"type\":\"ConnectorPlacement.EquallySpacedRectSide\",\"uuid\":\"a0066dd6-a193-491c-afbe-bac00dfc3505\"}]},\"type\":\"ConnectorPlacement.EquallySpacedConnector\",\"uuid\":\"c80211c6-bb24-481b-97ca-2752015f3b18\"}],\"packageUris\":[\"http://schema.mathworks.com/mf0/Connector/19700101\"],\"version\":\"1.0\"}"
  Tile26 : Subsystem  mask(Square Tile){side=side, thickness=thick, color=color2, opacity=opacity}
      mask prompts: side "Side (m) :"; thickness "Thickness (m) :"; color "Color [RGB] :"; opacity "Opacity (0...1) :"
      mask help: This block creates a flat, single, square tile element. The square tile body is mass-less, so it will not have an effect on the dynamic simulation. This square tile element can be used as a graphic reference by itself, or as part of a composite graphic reference made of an array of interconnected tiles. The square tile is aligned with the XY plane, and the block provides frame connector ports to the middle points on each of the four sides of the body of the square - right (+X), left (-X), top (+Y) and bottom (-Y). All dimensions are in meters.
      settings: PortSchema="{\"entries\":[{\"content\":{\"sides\":[{\"content\":{\"connectorIds\":[\"LConn1\"]},\"type\":\"ConnectorPlacement.EquallySpacedRectSide\",\"uuid\":\"a971723f-ea37-4e9b-910b-501b94fb0ba2\"},{\"content\":{\"connectorIds\":[\"RConn1\"],\"side\":\"RIGHT\"},\"type\":\"ConnectorPlacement.EquallySpacedRectSide\",\"uuid\":\"e50175c1-005c-4b0b-bced-b882197eaab2\"},{\"content\":{\"connectorIds\":[\"LConn2\"],\"side\":\"TOP\"},\"type\":\"ConnectorPlacement.EquallySpacedRectSide\",\"uuid\":\"2a04a964-d53e-47ee-8c79-d53dd599bafe\"},{\"content\":{\"connectorIds\":[\"RConn2\"],\"side\":\"BOTTOM\"},\"type\":\"ConnectorPlacement.EquallySpacedRectSide\",\"uuid\":\"a0066dd6-a193-491c-afbe-bac00dfc3505\"}]},\"type\":\"ConnectorPlacement.EquallySpacedConnector\",\"uuid\":\"c80211c6-bb24-481b-97ca-2752015f3b18\"}],\"packageUris\":[\"http://schema.mathworks.com/mf0/Connector/19700101\"],\"version\":\"1.0\"}"
  Tile27 : Subsystem  mask(Square Tile){side=side, thickness=thick, color=color1, opacity=opacity}
      mask prompts: side "Side (m) :"; thickness "Thickness (m) :"; color "Color [RGB] :"; opacity "Opacity (0...1) :"
      mask help: This block creates a flat, single, square tile element. The square tile body is mass-less, so it will not have an effect on the dynamic simulation. This square tile element can be used as a graphic reference by itself, or as part of a composite graphic reference made of an array of interconnected tiles. The square tile is aligned with the XY plane, and the block provides frame connector ports to the middle points on each of the four sides of the body of the square - right (+X), left (-X), top (+Y) and bottom (-Y). All dimensions are in meters.
      settings: PortSchema="{\"entries\":[{\"content\":{\"sides\":[{\"content\":{\"connectorIds\":[\"LConn1\"]},\"type\":\"ConnectorPlacement.EquallySpacedRectSide\",\"uuid\":\"a971723f-ea37-4e9b-910b-501b94fb0ba2\"},{\"content\":{\"connectorIds\":[\"RConn1\"],\"side\":\"RIGHT\"},\"type\":\"ConnectorPlacement.EquallySpacedRectSide\",\"uuid\":\"e50175c1-005c-4b0b-bced-b882197eaab2\"},{\"content\":{\"connectorIds\":[\"LConn2\"],\"side\":\"TOP\"},\"type\":\"ConnectorPlacement.EquallySpacedRectSide\",\"uuid\":\"2a04a964-d53e-47ee-8c79-d53dd599bafe\"},{\"content\":{\"connectorIds\":[\"RConn2\"],\"side\":\"BOTTOM\"},\"type\":\"ConnectorPlacement.EquallySpacedRectSide\",\"uuid\":\"a0066dd6-a193-491c-afbe-bac00dfc3505\"}]},\"type\":\"ConnectorPlacement.EquallySpacedConnector\",\"uuid\":\"c80211c6-bb24-481b-97ca-2752015f3b18\"}],\"packageUris\":[\"http://schema.mathworks.com/mf0/Connector/19700101\"],\"version\":\"1.0\"}"
  Tile28 : Subsystem  mask(Square Tile){side=side, thickness=thick, color=color2, opacity=opacity}
      mask prompts: side "Side (m) :"; thickness "Thickness (m) :"; color "Color [RGB] :"; opacity "Opacity (0...1) :"
      mask help: This block creates a flat, single, square tile element. The square tile body is mass-less, so it will not have an effect on the dynamic simulation. This square tile element can be used as a graphic reference by itself, or as part of a composite graphic reference made of an array of interconnected tiles. The square tile is aligned with the XY plane, and the block provides frame connector ports to the middle points on each of the four sides of the body of the square - right (+X), left (-X), top (+Y) and bottom (-Y). All dimensions are in meters.
      settings: PortSchema="{\"entries\":[{\"content\":{\"sides\":[{\"content\":{\"connectorIds\":[\"LConn1\"]},\"type\":\"ConnectorPlacement.EquallySpacedRectSide\",\"uuid\":\"a971723f-ea37-4e9b-910b-501b94fb0ba2\"},{\"content\":{\"connectorIds\":[\"RConn1\"],\"side\":\"RIGHT\"},\"type\":\"ConnectorPlacement.EquallySpacedRectSide\",\"uuid\":\"e50175c1-005c-4b0b-bced-b882197eaab2\"},{\"content\":{\"connectorIds\":[\"LConn2\"],\"side\":\"TOP\"},\"type\":\"ConnectorPlacement.EquallySpacedRectSide\",\"uuid\":\"2a04a964-d53e-47ee-8c79-d53dd599bafe\"},{\"content\":{\"connectorIds\":[\"RConn2\"],\"side\":\"BOTTOM\"},\"type\":\"ConnectorPlacement.EquallySpacedRectSide\",\"uuid\":\"a0066dd6-a193-491c-afbe-bac00dfc3505\"}]},\"type\":\"ConnectorPlacement.EquallySpacedConnector\",\"uuid\":\"c80211c6-bb24-481b-97ca-2752015f3b18\"}],\"packageUris\":[\"http://schema.mathworks.com/mf0/Connector/19700101\"],\"version\":\"1.0\"}"
  Tile29 : Subsystem  mask(Square Tile){side=side, thickness=thick, color=color1, opacity=opacity}
      mask prompts: side "Side (m) :"; thickness "Thickness (m) :"; color "Color [RGB] :"; opacity "Opacity (0...1) :"
      mask help: This block creates a flat, single, square tile element. The square tile body is mass-less, so it will not have an effect on the dynamic simulation. This square tile element can be used as a graphic reference by itself, or as part of a composite graphic reference made of an array of interconnected tiles. The square tile is aligned with the XY plane, and the block provides frame connector ports to the middle points on each of the four sides of the body of the square - right (+X), left (-X), top (+Y) and bottom (-Y). All dimensions are in meters.
      settings: PortSchema="{\"entries\":[{\"content\":{\"sides\":[{\"content\":{\"connectorIds\":[\"LConn1\"]},\"type\":\"ConnectorPlacement.EquallySpacedRectSide\",\"uuid\":\"a971723f-ea37-4e9b-910b-501b94fb0ba2\"},{\"content\":{\"connectorIds\":[\"RConn1\"],\"side\":\"RIGHT\"},\"type\":\"ConnectorPlacement.EquallySpacedRectSide\",\"uuid\":\"e50175c1-005c-4b0b-bced-b882197eaab2\"},{\"content\":{\"connectorIds\":[\"LConn2\"],\"side\":\"TOP\"},\"type\":\"ConnectorPlacement.EquallySpacedRectSide\",\"uuid\":\"2a04a964-d53e-47ee-8c79-d53dd599bafe\"},{\"content\":{\"connectorIds\":[\"RConn2\"],\"side\":\"BOTTOM\"},\"type\":\"ConnectorPlacement.EquallySpacedRectSide\",\"uuid\":\"a0066dd6-a193-491c-afbe-bac00dfc3505\"}]},\"type\":\"ConnectorPlacement.EquallySpacedConnector\",\"uuid\":\"c80211c6-bb24-481b-97ca-2752015f3b18\"}],\"packageUris\":[\"http://schema.mathworks.com/mf0/Connector/19700101\"],\"version\":\"1.0\"}"
  Tile3 : Subsystem  mask(Square Tile){side=side, thickness=thick, color=color1, opacity=opacity}
      mask prompts: side "Side (m) :"; thickness "Thickness (m) :"; color "Color [RGB] :"; opacity "Opacity (0...1) :"
      mask help: This block creates a flat, single, square tile element. The square tile body is mass-less, so it will not have an effect on the dynamic simulation. This square tile element can be used as a graphic reference by itself, or as part of a composite graphic reference made of an array of interconnected tiles. The square tile is aligned with the XY plane, and the block provides frame connector ports to the middle points on each of the four sides of the body of the square - right (+X), left (-X), top (+Y) and bottom (-Y). All dimensions are in meters.
      settings: PortSchema="{\"entries\":[{\"content\":{\"sides\":[{\"content\":{\"connectorIds\":[\"LConn1\"]},\"type\":\"ConnectorPlacement.EquallySpacedRectSide\",\"uuid\":\"a971723f-ea37-4e9b-910b-501b94fb0ba2\"},{\"content\":{\"connectorIds\":[\"RConn1\"],\"side\":\"RIGHT\"},\"type\":\"ConnectorPlacement.EquallySpacedRectSide\",\"uuid\":\"e50175c1-005c-4b0b-bced-b882197eaab2\"},{\"content\":{\"connectorIds\":[\"LConn2\"],\"side\":\"TOP\"},\"type\":\"ConnectorPlacement.EquallySpacedRectSide\",\"uuid\":\"2a04a964-d53e-47ee-8c79-d53dd599bafe\"},{\"content\":{\"connectorIds\":[\"RConn2\"],\"side\":\"BOTTOM\"},\"type\":\"ConnectorPlacement.EquallySpacedRectSide\",\"uuid\":\"a0066dd6-a193-491c-afbe-bac00dfc3505\"}]},\"type\":\"ConnectorPlacement.EquallySpacedConnector\",\"uuid\":\"c80211c6-bb24-481b-97ca-2752015f3b18\"}],\"packageUris\":[\"http://schema.mathworks.com/mf0/Connector/19700101\"],\"version\":\"1.0\"}"
  Tile30 : Subsystem  mask(Square Tile){side=side, thickness=thick, color=color2, opacity=opacity}
      mask prompts: side "Side (m) :"; thickness "Thickness (m) :"; color "Color [RGB] :"; opacity "Opacity (0...1) :"
      mask help: This block creates a flat, single, square tile element. The square tile body is mass-less, so it will not have an effect on the dynamic simulation. This square tile element can be used as a graphic reference by itself, or as part of a composite graphic reference made of an array of interconnected tiles. The square tile is aligned with the XY plane, and the block provides frame connector ports to the middle points on each of the four sides of the body of the square - right (+X), left (-X), top (+Y) and bottom (-Y). All dimensions are in meters.
      settings: PortSchema="{\"entries\":[{\"content\":{\"sides\":[{\"content\":{\"connectorIds\":[\"LConn1\"]},\"type\":\"ConnectorPlacement.EquallySpacedRectSide\",\"uuid\":\"a971723f-ea37-4e9b-910b-501b94fb0ba2\"},{\"content\":{\"connectorIds\":[\"RConn1\"],\"side\":\"RIGHT\"},\"type\":\"ConnectorPlacement.EquallySpacedRectSide\",\"uuid\":\"e50175c1-005c-4b0b-bced-b882197eaab2\"},{\"content\":{\"connectorIds\":[\"LConn2\"],\"side\":\"TOP\"},\"type\":\"ConnectorPlacement.EquallySpacedRectSide\",\"uuid\":\"2a04a964-d53e-47ee-8c79-d53dd599bafe\"},{\"content\":{\"connectorIds\":[\"RConn2\"],\"side\":\"BOTTOM\"},\"type\":\"ConnectorPlacement.EquallySpacedRectSide\",\"uuid\":\"a0066dd6-a193-491c-afbe-bac00dfc3505\"}]},\"type\":\"ConnectorPlacement.EquallySpacedConnector\",\"uuid\":\"c80211c6-bb24-481b-97ca-2752015f3b18\"}],\"packageUris\":[\"http://schema.mathworks.com/mf0/Connector/19700101\"],\"version\":\"1.0\"}"
  Tile31 : Subsystem  mask(Square Tile){side=side, thickness=thick, color=color1, opacity=opacity}
      mask prompts: side "Side (m) :"; thickness "Thickness (m) :"; color "Color [RGB] :"; opacity "Opacity (0...1) :"
      mask help: This block creates a flat, single, square tile element. The square tile body is mass-less, so it will not have an effect on the dynamic simulation. This square tile element can be used as a graphic reference by itself, or as part of a composite graphic reference made of an array of interconnected tiles. The square tile is aligned with the XY plane, and the block provides frame connector ports to the middle points on each of the four sides of the body of the square - right (+X), left (-X), top (+Y) and bottom (-Y). All dimensions are in meters.
      settings: PortSchema="{\"entries\":[{\"content\":{\"sides\":[{\"content\":{\"connectorIds\":[\"LConn1\"]},\"type\":\"ConnectorPlacement.EquallySpacedRectSide\",\"uuid\":\"a971723f-ea37-4e9b-910b-501b94fb0ba2\"},{\"content\":{\"connectorIds\":[\"RConn1\"],\"side\":\"RIGHT\"},\"type\":\"ConnectorPlacement.EquallySpacedRectSide\",\"uuid\":\"e50175c1-005c-4b0b-bced-b882197eaab2\"},{\"content\":{\"connectorIds\":[\"LConn2\"],\"side\":\"TOP\"},\"type\":\"ConnectorPlacement.EquallySpacedRectSide\",\"uuid\":\"2a04a964-d53e-47ee-8c79-d53dd599bafe\"},{\"content\":{\"connectorIds\":[\"RConn2\"],\"side\":\"BOTTOM\"},\"type\":\"ConnectorPlacement.EquallySpacedRectSide\",\"uuid\":\"a0066dd6-a193-491c-afbe-bac00dfc3505\"}]},\"type\":\"ConnectorPlacement.EquallySpacedConnector\",\"uuid\":\"c80211c6-bb24-481b-97ca-2752015f3b18\"}],\"packageUris\":[\"http://schema.mathworks.com/mf0/Connector/19700101\"],\"version\":\"1.0\"}"
  Tile32 : Subsystem  mask(Square Tile){side=side, thickness=thick, color=color2, opacity=opacity}
      mask prompts: side "Side (m) :"; thickness "Thickness (m) :"; color "Color [RGB] :"; opacity "Opacity (0...1) :"
      mask help: This block creates a flat, single, square tile element. The square tile body is mass-less, so it will not have an effect on the dynamic simulation. This square tile element can be used as a graphic reference by itself, or as part of a composite graphic reference made of an array of interconnected tiles. The square tile is aligned with the XY plane, and the block provides frame connector ports to the middle points on each of the four sides of the body of the square - right (+X), left (-X), top (+Y) and bottom (-Y). All dimensions are in meters.
      settings: PortSchema="{\"entries\":[{\"content\":{\"sides\":[{\"content\":{\"connectorIds\":[\"LConn1\"]},\"type\":\"ConnectorPlacement.EquallySpacedRectSide\",\"uuid\":\"a971723f-ea37-4e9b-910b-501b94fb0ba2\"},{\"content\":{\"connectorIds\":[\"RConn1\"],\"side\":\"RIGHT\"},\"type\":\"ConnectorPlacement.EquallySpacedRectSide\",\"uuid\":\"e50175c1-005c-4b0b-bced-b882197eaab2\"},{\"content\":{\"connectorIds\":[\"LConn2\"],\"side\":\"TOP\"},\"type\":\"ConnectorPlacement.EquallySpacedRectSide\",\"uuid\":\"2a04a964-d53e-47ee-8c79-d53dd599bafe\"},{\"content\":{\"connectorIds\":[\"RConn2\"],\"side\":\"BOTTOM\"},\"type\":\"ConnectorPlacement.EquallySpacedRectSide\",\"uuid\":\"a0066dd6-a193-491c-afbe-bac00dfc3505\"}]},\"type\":\"ConnectorPlacement.EquallySpacedConnector\",\"uuid\":\"c80211c6-bb24-481b-97ca-2752015f3b18\"}],\"packageUris\":[\"http://schema.mathworks.com/mf0/Connector/19700101\"],\"version\":\"1.0\"}"
  Tile33 : Subsystem  mask(Square Tile){side=side, thickness=thick, color=color1, opacity=opacity}
      mask prompts: side "Side (m) :"; thickness "Thickness (m) :"; color "Color [RGB] :"; opacity "Opacity (0...1) :"
      mask help: This block creates a flat, single, square tile element. The square tile body is mass-less, so it will not have an effect on the dynamic simulation. This square tile element can be used as a graphic reference by itself, or as part of a composite graphic reference made of an array of interconnected tiles. The square tile is aligned with the XY plane, and the block provides frame connector ports to the middle points on each of the four sides of the body of the square - right (+X), left (-X), top (+Y) and bottom (-Y). All dimensions are in meters.
      settings: PortSchema="{\"entries\":[{\"content\":{\"sides\":[{\"content\":{\"connectorIds\":[\"LConn1\"]},\"type\":\"ConnectorPlacement.EquallySpacedRectSide\",\"uuid\":\"a971723f-ea37-4e9b-910b-501b94fb0ba2\"},{\"content\":{\"connectorIds\":[\"RConn1\"],\"side\":\"RIGHT\"},\"type\":\"ConnectorPlacement.EquallySpacedRectSide\",\"uuid\":\"e50175c1-005c-4b0b-bced-b882197eaab2\"},{\"content\":{\"connectorIds\":[\"LConn2\"],\"side\":\"TOP\"},\"type\":\"ConnectorPlacement.EquallySpacedRectSide\",\"uuid\":\"2a04a964-d53e-47ee-8c79-d53dd599bafe\"},{\"content\":{\"connectorIds\":[\"RConn2\"],\"side\":\"BOTTOM\"},\"type\":\"ConnectorPlacement.EquallySpacedRectSide\",\"uuid\":\"a0066dd6-a193-491c-afbe-bac00dfc3505\"}]},\"type\":\"ConnectorPlacement.EquallySpacedConnector\",\"uuid\":\"c80211c6-bb24-481b-97ca-2752015f3b18\"}],\"packageUris\":[\"http://schema.mathworks.com/mf0/Connector/19700101\"],\"version\":\"1.0\"}"
  Tile34 : Subsystem  mask(Square Tile){side=side, thickness=thick, color=color1, opacity=opacity}
      mask prompts: side "Side (m) :"; thickness "Thickness (m) :"; color "Color [RGB] :"; opacity "Opacity (0...1) :"
      mask help: This block creates a flat, single, square tile element. The square tile body is mass-less, so it will not have an effect on the dynamic simulation. This square tile element can be used as a graphic reference by itself, or as part of a composite graphic reference made of an array of interconnected tiles. The square tile is aligned with the XY plane, and the block provides frame connector ports to the middle points on each of the four sides of the body of the square - right (+X), left (-X), top (+Y) and bottom (-Y). All dimensions are in meters.
      settings: PortSchema="{\"entries\":[{\"content\":{\"sides\":[{\"content\":{\"connectorIds\":[\"LConn1\"]},\"type\":\"ConnectorPlacement.EquallySpacedRectSide\",\"uuid\":\"a971723f-ea37-4e9b-910b-501b94fb0ba2\"},{\"content\":{\"connectorIds\":[\"RConn1\"],\"side\":\"RIGHT\"},\"type\":\"ConnectorPlacement.EquallySpacedRectSide\",\"uuid\":\"e50175c1-005c-4b0b-bced-b882197eaab2\"},{\"content\":{\"connectorIds\":[\"LConn2\"],\"side\":\"TOP\"},\"type\":\"ConnectorPlacement.EquallySpacedRectSide\",\"uuid\":\"2a04a964-d53e-47ee-8c79-d53dd599bafe\"},{\"content\":{\"connectorIds\":[\"RConn2\"],\"side\":\"BOTTOM\"},\"type\":\"ConnectorPlacement.EquallySpacedRectSide\",\"uuid\":\"a0066dd6-a193-491c-afbe-bac00dfc3505\"}]},\"type\":\"ConnectorPlacement.EquallySpacedConnector\",\"uuid\":\"c80211c6-bb24-481b-97ca-2752015f3b18\"}],\"packageUris\":[\"http://schema.mathworks.com/mf0/Connector/19700101\"],\"version\":\"1.0\"}"
  Tile35 : Subsystem  mask(Square Tile){side=side, thickness=thick, color=color2, opacity=opacity}
      mask prompts: side "Side (m) :"; thickness "Thickness (m) :"; color "Color [RGB] :"; opacity "Opacity (0...1) :"
      mask help: This block creates a flat, single, square tile element. The square tile body is mass-less, so it will not have an effect on the dynamic simulation. This square tile element can be used as a graphic reference by itself, or as part of a composite graphic reference made of an array of interconnected tiles. The square tile is aligned with the XY plane, and the block provides frame connector ports to the middle points on each of the four sides of the body of the square - right (+X), left (-X), top (+Y) and bottom (-Y). All dimensions are in meters.
      settings: PortSchema="{\"entries\":[{\"content\":{\"sides\":[{\"content\":{\"connectorIds\":[\"LConn1\"]},\"type\":\"ConnectorPlacement.EquallySpacedRectSide\",\"uuid\":\"a971723f-ea37-4e9b-910b-501b94fb0ba2\"},{\"content\":{\"connectorIds\":[\"RConn1\"],\"side\":\"RIGHT\"},\"type\":\"ConnectorPlacement.EquallySpacedRectSide\",\"uuid\":\"e50175c1-005c-4b0b-bced-b882197eaab2\"},{\"content\":{\"connectorIds\":[\"LConn2\"],\"side\":\"TOP\"},\"type\":\"ConnectorPlacement.EquallySpacedRectSide\",\"uuid\":\"2a04a964-d53e-47ee-8c79-d53dd599bafe\"},{\"content\":{\"connectorIds\":[\"RConn2\"],\"side\":\"BOTTOM\"},\"type\":\"ConnectorPlacement.EquallySpacedRectSide\",\"uuid\":\"a0066dd6-a193-491c-afbe-bac00dfc3505\"}]},\"type\":\"ConnectorPlacement.EquallySpacedConnector\",\"uuid\":\"c80211c6-bb24-481b-97ca-2752015f3b18\"}],\"packageUris\":[\"http://schema.mathworks.com/mf0/Connector/19700101\"],\"version\":\"1.0\"}"
  Tile36 : Subsystem  mask(Square Tile){side=side, thickness=thick, color=color1, opacity=opacity}
      mask prompts: side "Side (m) :"; thickness "Thickness (m) :"; color "Color [RGB] :"; opacity "Opacity (0...1) :"
      mask help: This block creates a flat, single, square tile element. The square tile body is mass-less, so it will not have an effect on the dynamic simulation. This square tile element can be used as a graphic reference by itself, or as part of a composite graphic reference made of an array of interconnected tiles. The square tile is aligned with the XY plane, and the block provides frame connector ports to the middle points on each of the four sides of the body of the square - right (+X), left (-X), top (+Y) and bottom (-Y). All dimensions are in meters.
      settings: PortSchema="{\"entries\":[{\"content\":{\"sides\":[{\"content\":{\"connectorIds\":[\"LConn1\"]},\"type\":\"ConnectorPlacement.EquallySpacedRectSide\",\"uuid\":\"a971723f-ea37-4e9b-910b-501b94fb0ba2\"},{\"content\":{\"connectorIds\":[\"RConn1\"],\"side\":\"RIGHT\"},\"type\":\"ConnectorPlacement.EquallySpacedRectSide\",\"uuid\":\"e50175c1-005c-4b0b-bced-b882197eaab2\"},{\"content\":{\"connectorIds\":[\"LConn2\"],\"side\":\"TOP\"},\"type\":\"ConnectorPlacement.EquallySpacedRectSide\",\"uuid\":\"2a04a964-d53e-47ee-8c79-d53dd599bafe\"},{\"content\":{\"connectorIds\":[\"RConn2\"],\"side\":\"BOTTOM\"},\"type\":\"ConnectorPlacement.EquallySpacedRectSide\",\"uuid\":\"a0066dd6-a193-491c-afbe-bac00dfc3505\"}]},\"type\":\"ConnectorPlacement.EquallySpacedConnector\",\"uuid\":\"c80211c6-bb24-481b-97ca-2752015f3b18\"}],\"packageUris\":[\"http://schema.mathworks.com/mf0/Connector/19700101\"],\"version\":\"1.0\"}"
  Tile37 : Subsystem  mask(Square Tile){side=side, thickness=thick, color=color2, opacity=opacity}
      mask prompts: side "Side (m) :"; thickness "Thickness (m) :"; color "Color [RGB] :"; opacity "Opacity (0...1) :"
      mask help: This block creates a flat, single, square tile element. The square tile body is mass-less, so it will not have an effect on the dynamic simulation. This square tile element can be used as a graphic reference by itself, or as part of a composite graphic reference made of an array of interconnected tiles. The square tile is aligned with the XY plane, and the block provides frame connector ports to the middle points on each of the four sides of the body of the square - right (+X), left (-X), top (+Y) and bottom (-Y). All dimensions are in meters.
      settings: PortSchema="{\"entries\":[{\"content\":{\"sides\":[{\"content\":{\"connectorIds\":[\"LConn1\"]},\"type\":\"ConnectorPlacement.EquallySpacedRectSide\",\"uuid\":\"a971723f-ea37-4e9b-910b-501b94fb0ba2\"},{\"content\":{\"connectorIds\":[\"RConn1\"],\"side\":\"RIGHT\"},\"type\":\"ConnectorPlacement.EquallySpacedRectSide\",\"uuid\":\"e50175c1-005c-4b0b-bced-b882197eaab2\"},{\"content\":{\"connectorIds\":[\"LConn2\"],\"side\":\"TOP\"},\"type\":\"ConnectorPlacement.EquallySpacedRectSide\",\"uuid\":\"2a04a964-d53e-47ee-8c79-d53dd599bafe\"},{\"content\":{\"connectorIds\":[\"RConn2\"],\"side\":\"BOTTOM\"},\"type\":\"ConnectorPlacement.EquallySpacedRectSide\",\"uuid\":\"a0066dd6-a193-491c-afbe-bac00dfc3505\"}]},\"type\":\"ConnectorPlacement.EquallySpacedConnector\",\"uuid\":\"c80211c6-bb24-481b-97ca-2752015f3b18\"}],\"packageUris\":[\"http://schema.mathworks.com/mf0/Connector/19700101\"],\"version\":\"1.0\"}"
  Tile38 : Subsystem  mask(Square Tile){side=side, thickness=thick, color=color1, opacity=opacity}
      mask prompts: side "Side (m) :"; thickness "Thickness (m) :"; color "Color [RGB] :"; opacity "Opacity (0...1) :"
      mask help: This block creates a flat, single, square tile element. The square tile body is mass-less, so it will not have an effect on the dynamic simulation. This square tile element can be used as a graphic reference by itself, or as part of a composite graphic reference made of an array of interconnected tiles. The square tile is aligned with the XY plane, and the block provides frame connector ports to the middle points on each of the four sides of the body of the square - right (+X), left (-X), top (+Y) and bottom (-Y). All dimensions are in meters.
      settings: PortSchema="{\"entries\":[{\"content\":{\"sides\":[{\"content\":{\"connectorIds\":[\"LConn1\"]},\"type\":\"ConnectorPlacement.EquallySpacedRectSide\",\"uuid\":\"a971723f-ea37-4e9b-910b-501b94fb0ba2\"},{\"content\":{\"connectorIds\":[\"RConn1\"],\"side\":\"RIGHT\"},\"type\":\"ConnectorPlacement.EquallySpacedRectSide\",\"uuid\":\"e50175c1-005c-4b0b-bced-b882197eaab2\"},{\"content\":{\"connectorIds\":[\"LConn2\"],\"side\":\"TOP\"},\"type\":\"ConnectorPlacement.EquallySpacedRectSide\",\"uuid\":\"2a04a964-d53e-47ee-8c79-d53dd599bafe\"},{\"content\":{\"connectorIds\":[\"RConn2\"],\"side\":\"BOTTOM\"},\"type\":\"ConnectorPlacement.EquallySpacedRectSide\",\"uuid\":\"a0066dd6-a193-491c-afbe-bac00dfc3505\"}]},\"type\":\"ConnectorPlacement.EquallySpacedConnector\",\"uuid\":\"c80211c6-bb24-481b-97ca-2752015f3b18\"}],\"packageUris\":[\"http://schema.mathworks.com/mf0/Connector/19700101\"],\"version\":\"1.0\"}"
  Tile39 : Subsystem  mask(Square Tile){side=side, thickness=thick, color=color2, opacity=opacity}
      mask prompts: side "Side (m) :"; thickness "Thickness (m) :"; color "Color [RGB] :"; opacity "Opacity (0...1) :"
      mask help: This block creates a flat, single, square tile element. The square tile body is mass-less, so it will not have an effect on the dynamic simulation. This square tile element can be used as a graphic reference by itself, or as part of a composite graphic reference made of an array of interconnected tiles. The square tile is aligned with the XY plane, and the block provides frame connector ports to the middle points on each of the four sides of the body of the square - right (+X), left (-X), top (+Y) and bottom (-Y). All dimensions are in meters.
      settings: PortSchema="{\"entries\":[{\"content\":{\"sides\":[{\"content\":{\"connectorIds\":[\"LConn1\"]},\"type\":\"ConnectorPlacement.EquallySpacedRectSide\",\"uuid\":\"a971723f-ea37-4e9b-910b-501b94fb0ba2\"},{\"content\":{\"connectorIds\":[\"RConn1\"],\"side\":\"RIGHT\"},\"type\":\"ConnectorPlacement.EquallySpacedRectSide\",\"uuid\":\"e50175c1-005c-4b0b-bced-b882197eaab2\"},{\"content\":{\"connectorIds\":[\"LConn2\"],\"side\":\"TOP\"},\"type\":\"ConnectorPlacement.EquallySpacedRectSide\",\"uuid\":\"2a04a964-d53e-47ee-8c79-d53dd599bafe\"},{\"content\":{\"connectorIds\":[\"RConn2\"],\"side\":\"BOTTOM\"},\"type\":\"ConnectorPlacement.EquallySpacedRectSide\",\"uuid\":\"a0066dd6-a193-491c-afbe-bac00dfc3505\"}]},\"type\":\"ConnectorPlacement.EquallySpacedConnector\",\"uuid\":\"c80211c6-bb24-481b-97ca-2752015f3b18\"}],\"packageUris\":[\"http://schema.mathworks.com/mf0/Connector/19700101\"],\"version\":\"1.0\"}"
  Tile4 : Subsystem  mask(Square Tile){side=side, thickness=thick, color=color2, opacity=opacity}
      mask prompts: side "Side (m) :"; thickness "Thickness (m) :"; color "Color [RGB] :"; opacity "Opacity (0...1) :"
      mask help: This block creates a flat, single, square tile element. The square tile body is mass-less, so it will not have an effect on the dynamic simulation. This square tile element can be used as a graphic reference by itself, or as part of a composite graphic reference made of an array of interconnected tiles. The square tile is aligned with the XY plane, and the block provides frame connector ports to the middle points on each of the four sides of the body of the square - right (+X), left (-X), top (+Y) and bottom (-Y). All dimensions are in meters.
      settings: PortSchema="{\"entries\":[{\"content\":{\"sides\":[{\"content\":{\"connectorIds\":[\"LConn1\"]},\"type\":\"ConnectorPlacement.EquallySpacedRectSide\",\"uuid\":\"a971723f-ea37-4e9b-910b-501b94fb0ba2\"},{\"content\":{\"connectorIds\":[\"RConn1\"],\"side\":\"RIGHT\"},\"type\":\"ConnectorPlacement.EquallySpacedRectSide\",\"uuid\":\"e50175c1-005c-4b0b-bced-b882197eaab2\"},{\"content\":{\"connectorIds\":[\"LConn2\"],\"side\":\"TOP\"},\"type\":\"ConnectorPlacement.EquallySpacedRectSide\",\"uuid\":\"2a04a964-d53e-47ee-8c79-d53dd599bafe\"},{\"content\":{\"connectorIds\":[\"RConn2\"],\"side\":\"BOTTOM\"},\"type\":\"ConnectorPlacement.EquallySpacedRectSide\",\"uuid\":\"a0066dd6-a193-491c-afbe-bac00dfc3505\"}]},\"type\":\"ConnectorPlacement.EquallySpacedConnector\",\"uuid\":\"c80211c6-bb24-481b-97ca-2752015f3b18\"}],\"packageUris\":[\"http://schema.mathworks.com/mf0/Connector/19700101\"],\"version\":\"1.0\"}"
  Tile40 : Subsystem  mask(Square Tile){side=side, thickness=thick, color=color1, opacity=opacity}
      mask prompts: side "Side (m) :"; thickness "Thickness (m) :"; color "Color [RGB] :"; opacity "Opacity (0...1) :"
      mask help: This block creates a flat, single, square tile element. The square tile body is mass-less, so it will not have an effect on the dynamic simulation. This square tile element can be used as a graphic reference by itself, or as part of a composite graphic reference made of an array of interconnected tiles. The square tile is aligned with the XY plane, and the block provides frame connector ports to the middle points on each of the four sides of the body of the square - right (+X), left (-X), top (+Y) and bottom (-Y). All dimensions are in meters.
      settings: PortSchema="{\"entries\":[{\"content\":{\"sides\":[{\"content\":{\"connectorIds\":[\"LConn1\"]},\"type\":\"ConnectorPlacement.EquallySpacedRectSide\",\"uuid\":\"a971723f-ea37-4e9b-910b-501b94fb0ba2\"},{\"content\":{\"connectorIds\":[\"RConn1\"],\"side\":\"RIGHT\"},\"type\":\"ConnectorPlacement.EquallySpacedRectSide\",\"uuid\":\"e50175c1-005c-4b0b-bced-b882197eaab2\"},{\"content\":{\"connectorIds\":[\"LConn2\"],\"side\":\"TOP\"},\"type\":\"ConnectorPlacement.EquallySpacedRectSide\",\"uuid\":\"2a04a964-d53e-47ee-8c79-d53dd599bafe\"},{\"content\":{\"connectorIds\":[\"RConn2\"],\"side\":\"BOTTOM\"},\"type\":\"ConnectorPlacement.EquallySpacedRectSide\",\"uuid\":\"a0066dd6-a193-491c-afbe-bac00dfc3505\"}]},\"type\":\"ConnectorPlacement.EquallySpacedConnector\",\"uuid\":\"c80211c6-bb24-481b-97ca-2752015f3b18\"}],\"packageUris\":[\"http://schema.mathworks.com/mf0/Connector/19700101\"],\"version\":\"1.0\"}"
  Tile41 : Subsystem  mask(Square Tile){side=side, thickness=thick, color=color1, opacity=opacity}
      mask prompts: side "Side (m) :"; thickness "Thickness (m) :"; color "Color [RGB] :"; opacity "Opacity (0...1) :"
      mask help: This block creates a flat, single, square tile element. The square tile body is mass-less, so it will not have an effect on the dynamic simulation. This square tile element can be used as a graphic reference by itself, or as part of a composite graphic reference made of an array of interconnected tiles. The square tile is aligned with the XY plane, and the block provides frame connector ports to the middle points on each of the four sides of the body of the square - right (+X), left (-X), top (+Y) and bottom (-Y). All dimensions are in meters.
      settings: PortSchema="{\"entries\":[{\"content\":{\"sides\":[{\"content\":{\"connectorIds\":[\"LConn1\"]},\"type\":\"ConnectorPlacement.EquallySpacedRectSide\",\"uuid\":\"a971723f-ea37-4e9b-910b-501b94fb0ba2\"},{\"content\":{\"connectorIds\":[\"RConn1\"],\"side\":\"RIGHT\"},\"type\":\"ConnectorPlacement.EquallySpacedRectSide\",\"uuid\":\"e50175c1-005c-4b0b-bced-b882197eaab2\"},{\"content\":{\"connectorIds\":[\"LConn2\"],\"side\":\"TOP\"},\"type\":\"ConnectorPlacement.EquallySpacedRectSide\",\"uuid\":\"2a04a964-d53e-47ee-8c79-d53dd599bafe\"},{\"content\":{\"connectorIds\":[\"RConn2\"],\"side\":\"BOTTOM\"},\"type\":\"ConnectorPlacement.EquallySpacedRectSide\",\"uuid\":\"a0066dd6-a193-491c-afbe-bac00dfc3505\"}]},\"type\":\"ConnectorPlacement.EquallySpacedConnector\",\"uuid\":\"c80211c6-bb24-481b-97ca-2752015f3b18\"}],\"packageUris\":[\"http://schema.mathworks.com/mf0/Connector/19700101\"],\"version\":\"1.0\"}"
  Tile42 : Subsystem  mask(Square Tile){side=side, thickness=thick, color=color2, opacity=opacity}
      mask prompts: side "Side (m) :"; thickness "Thickness (m) :"; color "Color [RGB] :"; opacity "Opacity (0...1) :"
      mask help: This block creates a flat, single, square tile element. The square tile body is mass-less, so it will not have an effect on the dynamic simulation. This square tile element can be used as a graphic reference by itself, or as part of a composite graphic reference made of an array of interconnected tiles. The square tile is aligned with the XY plane, and the block provides frame connector ports to the middle points on each of the four sides of the body of the square - right (+X), left (-X), top (+Y) and bottom (-Y). All dimensions are in meters.
      settings: PortSchema="{\"entries\":[{\"content\":{\"sides\":[{\"content\":{\"connectorIds\":[\"LConn1\"]},\"type\":\"ConnectorPlacement.EquallySpacedRectSide\",\"uuid\":\"a971723f-ea37-4e9b-910b-501b94fb0ba2\"},{\"content\":{\"connectorIds\":[\"RConn1\"],\"side\":\"RIGHT\"},\"type\":\"ConnectorPlacement.EquallySpacedRectSide\",\"uuid\":\"e50175c1-005c-4b0b-bced-b882197eaab2\"},{\"content\":{\"connectorIds\":[\"LConn2\"],\"side\":\"TOP\"},\"type\":\"ConnectorPlacement.EquallySpacedRectSide\",\"uuid\":\"2a04a964-d53e-47ee-8c79-d53dd599bafe\"},{\"content\":{\"connectorIds\":[\"RConn2\"],\"side\":\"BOTTOM\"},\"type\":\"ConnectorPlacement.EquallySpacedRectSide\",\"uuid\":\"a0066dd6-a193-491c-afbe-bac00dfc3505\"}]},\"type\":\"ConnectorPlacement.EquallySpacedConnector\",\"uuid\":\"c80211c6-bb24-481b-97ca-2752015f3b18\"}],\"packageUris\":[\"http://schema.mathworks.com/mf0/Connector/19700101\"],\"version\":\"1.0\"}"
  Tile43 : Subsystem  mask(Square Tile){side=side, thickness=thick, color=color2, opacity=opacity}
      mask prompts: side "Side (m) :"; thickness "Thickness (m) :"; color "Color [RGB] :"; opacity "Opacity (0...1) :"
      mask help: This block creates a flat, single, square tile element. The square tile body is mass-less, so it will not have an effect on the dynamic simulation. This square tile element can be used as a graphic reference by itself, or as part of a composite graphic reference made of an array of interconnected tiles. The square tile is aligned with the XY plane, and the block provides frame connector ports to the middle points on each of the four sides of the body of the square - right (+X), left (-X), top (+Y) and bottom (-Y). All dimensions are in meters.
      settings: PortSchema="{\"entries\":[{\"content\":{\"sides\":[{\"content\":{\"connectorIds\":[\"LConn1\"]},\"type\":\"ConnectorPlacement.EquallySpacedRectSide\",\"uuid\":\"a971723f-ea37-4e9b-910b-501b94fb0ba2\"},{\"content\":{\"connectorIds\":[\"RConn1\"],\"side\":\"RIGHT\"},\"type\":\"ConnectorPlacement.EquallySpacedRectSide\",\"uuid\":\"e50175c1-005c-4b0b-bced-b882197eaab2\"},{\"content\":{\"connectorIds\":[\"LConn2\"],\"side\":\"TOP\"},\"type\":\"ConnectorPlacement.EquallySpacedRectSide\",\"uuid\":\"2a04a964-d53e-47ee-8c79-d53dd599bafe\"},{\"content\":{\"connectorIds\":[\"RConn2\"],\"side\":\"BOTTOM\"},\"type\":\"ConnectorPlacement.EquallySpacedRectSide\",\"uuid\":\"a0066dd6-a193-491c-afbe-bac00dfc3505\"}]},\"type\":\"ConnectorPlacement.EquallySpacedConnector\",\"uuid\":\"c80211c6-bb24-481b-97ca-2752015f3b18\"}],\"packageUris\":[\"http://schema.mathworks.com/mf0/Connector/19700101\"],\"version\":\"1.0\"}"
  Tile44 : Subsystem  mask(Square Tile){side=side, thickness=thick, color=color1, opacity=opacity}
      mask prompts: side "Side (m) :"; thickness "Thickness (m) :"; color "Color [RGB] :"; opacity "Opacity (0...1) :"
      mask help: This block creates a flat, single, square tile element. The square tile body is mass-less, so it will not have an effect on the dynamic simulation. This square tile element can be used as a graphic reference by itself, or as part of a composite graphic reference made of an array of interconnected tiles. The square tile is aligned with the XY plane, and the block provides frame connector ports to the middle points on each of the four sides of the body of the square - right (+X), left (-X), top (+Y) and bottom (-Y). All dimensions are in meters.
      settings: PortSchema="{\"entries\":[{\"content\":{\"sides\":[{\"content\":{\"connectorIds\":[\"LConn1\"]},\"type\":\"ConnectorPlacement.EquallySpacedRectSide\",\"uuid\":\"a971723f-ea37-4e9b-910b-501b94fb0ba2\"},{\"content\":{\"connectorIds\":[\"RConn1\"],\"side\":\"RIGHT\"},\"type\":\"ConnectorPlacement.EquallySpacedRectSide\",\"uuid\":\"e50175c1-005c-4b0b-bced-b882197eaab2\"},{\"content\":{\"connectorIds\":[\"LConn2\"],\"side\":\"TOP\"},\"type\":\"ConnectorPlacement.EquallySpacedRectSide\",\"uuid\":\"2a04a964-d53e-47ee-8c79-d53dd599bafe\"},{\"content\":{\"connectorIds\":[\"RConn2\"],\"side\":\"BOTTOM\"},\"type\":\"ConnectorPlacement.EquallySpacedRectSide\",\"uuid\":\"a0066dd6-a193-491c-afbe-bac00dfc3505\"}]},\"type\":\"ConnectorPlacement.EquallySpacedConnector\",\"uuid\":\"c80211c6-bb24-481b-97ca-2752015f3b18\"}],\"packageUris\":[\"http://schema.mathworks.com/mf0/Connector/19700101\"],\"version\":\"1.0\"}"
  Tile45 : Subsystem  mask(Square Tile){side=side, thickness=thick, color=color2, opacity=opacity}
      mask prompts: side "Side (m) :"; thickness "Thickness (m) :"; color "Color [RGB] :"; opacity "Opacity (0...1) :"
      mask help: This block creates a flat, single, square tile element. The square tile body is mass-less, so it will not have an effect on the dynamic simulation. This square tile element can be used as a graphic reference by itself, or as part of a composite graphic reference made of an array of interconnected tiles. The square tile is aligned with the XY plane, and the block provides frame connector ports to the middle points on each of the four sides of the body of the square - right (+X), left (-X), top (+Y) and bottom (-Y). All dimensions are in meters.
      settings: PortSchema="{\"entries\":[{\"content\":{\"sides\":[{\"content\":{\"connectorIds\":[\"LConn1\"]},\"type\":\"ConnectorPlacement.EquallySpacedRectSide\",\"uuid\":\"a971723f-ea37-4e9b-910b-501b94fb0ba2\"},{\"content\":{\"connectorIds\":[\"RConn1\"],\"side\":\"RIGHT\"},\"type\":\"ConnectorPlacement.EquallySpacedRectSide\",\"uuid\":\"e50175c1-005c-4b0b-bced-b882197eaab2\"},{\"content\":{\"connectorIds\":[\"LConn2\"],\"side\":\"TOP\"},\"type\":\"ConnectorPlacement.EquallySpacedRectSide\",\"uuid\":\"2a04a964-d53e-47ee-8c79-d53dd599bafe\"},{\"content\":{\"connectorIds\":[\"RConn2\"],\"side\":\"BOTTOM\"},\"type\":\"ConnectorPlacement.EquallySpacedRectSide\",\"uuid\":\"a0066dd6-a193-491c-afbe-bac00dfc3505\"}]},\"type\":\"ConnectorPlacement.EquallySpacedConnector\",\"uuid\":\"c80211c6-bb24-481b-97ca-2752015f3b18\"}],\"packageUris\":[\"http://schema.mathworks.com/mf0/Connector/19700101\"],\"version\":\"1.0\"}"
  Tile46 : Subsystem  mask(Square Tile){side=side, thickness=thick, color=color1, opacity=opacity}
      mask prompts: side "Side (m) :"; thickness "Thickness (m) :"; color "Color [RGB] :"; opacity "Opacity (0...1) :"
      mask help: This block creates a flat, single, square tile element. The square tile body is mass-less, so it will not have an effect on the dynamic simulation. This square tile element can be used as a graphic reference by itself, or as part of a composite graphic reference made of an array of interconnected tiles. The square tile is aligned with the XY plane, and the block provides frame connector ports to the middle points on each of the four sides of the body of the square - right (+X), left (-X), top (+Y) and bottom (-Y). All dimensions are in meters.
      settings: PortSchema="{\"entries\":[{\"content\":{\"sides\":[{\"content\":{\"connectorIds\":[\"LConn1\"]},\"type\":\"ConnectorPlacement.EquallySpacedRectSide\",\"uuid\":\"a971723f-ea37-4e9b-910b-501b94fb0ba2\"},{\"content\":{\"connectorIds\":[\"RConn1\"],\"side\":\"RIGHT\"},\"type\":\"ConnectorPlacement.EquallySpacedRectSide\",\"uuid\":\"e50175c1-005c-4b0b-bced-b882197eaab2\"},{\"content\":{\"connectorIds\":[\"LConn2\"],\"side\":\"TOP\"},\"type\":\"ConnectorPlacement.EquallySpacedRectSide\",\"uuid\":\"2a04a964-d53e-47ee-8c79-d53dd599bafe\"},{\"content\":{\"connectorIds\":[\"RConn2\"],\"side\":\"BOTTOM\"},\"type\":\"ConnectorPlacement.EquallySpacedRectSide\",\"uuid\":\"a0066dd6-a193-491c-afbe-bac00dfc3505\"}]},\"type\":\"ConnectorPlacement.EquallySpacedConnector\",\"uuid\":\"c80211c6-bb24-481b-97ca-2752015f3b18\"}],\"packageUris\":[\"http://schema.mathworks.com/mf0/Connector/19700101\"],\"version\":\"1.0\"}"
  Tile47 : Subsystem  mask(Square Tile){side=side, thickness=thick, color=color2, opacity=opacity}
      mask prompts: side "Side (m) :"; thickness "Thickness (m) :"; color "Color [RGB] :"; opacity "Opacity (0...1) :"
      mask help: This block creates a flat, single, square tile element. The square tile body is mass-less, so it will not have an effect on the dynamic simulation. This square tile element can be used as a graphic reference by itself, or as part of a composite graphic reference made of an array of interconnected tiles. The square tile is aligned with the XY plane, and the block provides frame connector ports to the middle points on each of the four sides of the body of the square - right (+X), left (-X), top (+Y) and bottom (-Y). All dimensions are in meters.
      settings: PortSchema="{\"entries\":[{\"content\":{\"sides\":[{\"content\":{\"connectorIds\":[\"LConn1\"]},\"type\":\"ConnectorPlacement.EquallySpacedRectSide\",\"uuid\":\"a971723f-ea37-4e9b-910b-501b94fb0ba2\"},{\"content\":{\"connectorIds\":[\"RConn1\"],\"side\":\"RIGHT\"},\"type\":\"ConnectorPlacement.EquallySpacedRectSide\",\"uuid\":\"e50175c1-005c-4b0b-bced-b882197eaab2\"},{\"content\":{\"connectorIds\":[\"LConn2\"],\"side\":\"TOP\"},\"type\":\"ConnectorPlacement.EquallySpacedRectSide\",\"uuid\":\"2a04a964-d53e-47ee-8c79-d53dd599bafe\"},{\"content\":{\"connectorIds\":[\"RConn2\"],\"side\":\"BOTTOM\"},\"type\":\"ConnectorPlacement.EquallySpacedRectSide\",\"uuid\":\"a0066dd6-a193-491c-afbe-bac00dfc3505\"}]},\"type\":\"ConnectorPlacement.EquallySpacedConnector\",\"uuid\":\"c80211c6-bb24-481b-97ca-2752015f3b18\"}],\"packageUris\":[\"http://schema.mathworks.com/mf0/Connector/19700101\"],\"version\":\"1.0\"}"
  Tile48 : Subsystem  mask(Square Tile){side=side, thickness=thick, color=color1, opacity=opacity}
      mask prompts: side "Side (m) :"; thickness "Thickness (m) :"; color "Color [RGB] :"; opacity "Opacity (0...1) :"
      mask help: This block creates a flat, single, square tile element. The square tile body is mass-less, so it will not have an effect on the dynamic simulation. This square tile element can be used as a graphic reference by itself, or as part of a composite graphic reference made of an array of interconnected tiles. The square tile is aligned with the XY plane, and the block provides frame connector ports to the middle points on each of the four sides of the body of the square - right (+X), left (-X), top (+Y) and bottom (-Y). All dimensions are in meters.
      settings: PortSchema="{\"entries\":[{\"content\":{\"sides\":[{\"content\":{\"connectorIds\":[\"LConn1\"]},\"type\":\"ConnectorPlacement.EquallySpacedRectSide\",\"uuid\":\"a971723f-ea37-4e9b-910b-501b94fb0ba2\"},{\"content\":{\"connectorIds\":[\"RConn1\"],\"side\":\"RIGHT\"},\"type\":\"ConnectorPlacement.EquallySpacedRectSide\",\"uuid\":\"e50175c1-005c-4b0b-bced-b882197eaab2\"},{\"content\":{\"connectorIds\":[\"LConn2\"],\"side\":\"TOP\"},\"type\":\"ConnectorPlacement.EquallySpacedRectSide\",\"uuid\":\"2a04a964-d53e-47ee-8c79-d53dd599bafe\"},{\"content\":{\"connectorIds\":[\"RConn2\"],\"side\":\"BOTTOM\"},\"type\":\"ConnectorPlacement.EquallySpacedRectSide\",\"uuid\":\"a0066dd6-a193-491c-afbe-bac00dfc3505\"}]},\"type\":\"ConnectorPlacement.EquallySpacedConnector\",\"uuid\":\"c80211c6-bb24-481b-97ca-2752015f3b18\"}],\"packageUris\":[\"http://schema.mathworks.com/mf0/Connector/19700101\"],\"version\":\"1.0\"}"
  Tile49 : Subsystem  mask(Square Tile){side=side, thickness=thick, color=color2, opacity=opacity}
      mask prompts: side "Side (m) :"; thickness "Thickness (m) :"; color "Color [RGB] :"; opacity "Opacity (0...1) :"
      mask help: This block creates a flat, single, square tile element. The square tile body is mass-less, so it will not have an effect on the dynamic simulation. This square tile element can be used as a graphic reference by itself, or as part of a composite graphic reference made of an array of interconnected tiles. The square tile is aligned with the XY plane, and the block provides frame connector ports to the middle points on each of the four sides of the body of the square - right (+X), left (-X), top (+Y) and bottom (-Y). All dimensions are in meters.
      settings: PortSchema="{\"entries\":[{\"content\":{\"sides\":[{\"content\":{\"connectorIds\":[\"LConn1\"]},\"type\":\"ConnectorPlacement.EquallySpacedRectSide\",\"uuid\":\"a971723f-ea37-4e9b-910b-501b94fb0ba2\"},{\"content\":{\"connectorIds\":[\"RConn1\"],\"side\":\"RIGHT\"},\"type\":\"ConnectorPlacement.EquallySpacedRectSide\",\"uuid\":\"e50175c1-005c-4b0b-bced-b882197eaab2\"},{\"content\":{\"connectorIds\":[\"LConn2\"],\"side\":\"TOP\"},\"type\":\"ConnectorPlacement.EquallySpacedRectSide\",\"uuid\":\"2a04a964-d53e-47ee-8c79-d53dd599bafe\"},{\"content\":{\"connectorIds\":[\"RConn2\"],\"side\":\"BOTTOM\"},\"type\":\"ConnectorPlacement.EquallySpacedRectSide\",\"uuid\":\"a0066dd6-a193-491c-afbe-bac00dfc3505\"}]},\"type\":\"ConnectorPlacement.EquallySpacedConnector\",\"uuid\":\"c80211c6-bb24-481b-97ca-2752015f3b18\"}],\"packageUris\":[\"http://schema.mathworks.com/mf0/Connector/19700101\"],\"version\":\"1.0\"}"
  Tile5 : Subsystem  mask(Square Tile){side=side, thickness=thick, color=color1, opacity=opacity}
      mask prompts: side "Side (m) :"; thickness "Thickness (m) :"; color "Color [RGB] :"; opacity "Opacity (0...1) :"
      mask help: This block creates a flat, single, square tile element. The square tile body is mass-less, so it will not have an effect on the dynamic simulation. This square tile element can be used as a graphic reference by itself, or as part of a composite graphic reference made of an array of interconnected tiles. The square tile is aligned with the XY plane, and the block provides frame connector ports to the middle points on each of the four sides of the body of the square - right (+X), left (-X), top (+Y) and bottom (-Y). All dimensions are in meters.
      settings: PortSchema="{\"entries\":[{\"content\":{\"sides\":[{\"content\":{\"connectorIds\":[\"LConn1\"]},\"type\":\"ConnectorPlacement.EquallySpacedRectSide\",\"uuid\":\"a971723f-ea37-4e9b-910b-501b94fb0ba2\"},{\"content\":{\"connectorIds\":[\"RConn1\"],\"side\":\"RIGHT\"},\"type\":\"ConnectorPlacement.EquallySpacedRectSide\",\"uuid\":\"e50175c1-005c-4b0b-bced-b882197eaab2\"},{\"content\":{\"connectorIds\":[\"LConn2\"],\"side\":\"TOP\"},\"type\":\"ConnectorPlacement.EquallySpacedRectSide\",\"uuid\":\"2a04a964-d53e-47ee-8c79-d53dd599bafe\"},{\"content\":{\"connectorIds\":[\"RConn2\"],\"side\":\"BOTTOM\"},\"type\":\"ConnectorPlacement.EquallySpacedRectSide\",\"uuid\":\"a0066dd6-a193-491c-afbe-bac00dfc3505\"}]},\"type\":\"ConnectorPlacement.EquallySpacedConnector\",\"uuid\":\"c80211c6-bb24-481b-97ca-2752015f3b18\"}],\"packageUris\":[\"http://schema.mathworks.com/mf0/Connector/19700101\"],\"version\":\"1.0\"}"
  Tile50 : Subsystem  mask(Square Tile){side=side, thickness=thick, color=color1, opacity=opacity}
      mask prompts: side "Side (m) :"; thickness "Thickness (m) :"; color "Color [RGB] :"; opacity "Opacity (0...1) :"
      mask help: This block creates a flat, single, square tile element. The square tile body is mass-less, so it will not have an effect on the dynamic simulation. This square tile element can be used as a graphic reference by itself, or as part of a composite graphic reference made of an array of interconnected tiles. The square tile is aligned with the XY plane, and the block provides frame connector ports to the middle points on each of the four sides of the body of the square - right (+X), left (-X), top (+Y) and bottom (-Y). All dimensions are in meters.
      settings: PortSchema="{\"entries\":[{\"content\":{\"sides\":[{\"content\":{\"connectorIds\":[\"LConn1\"]},\"type\":\"ConnectorPlacement.EquallySpacedRectSide\",\"uuid\":\"a971723f-ea37-4e9b-910b-501b94fb0ba2\"},{\"content\":{\"connectorIds\":[\"RConn1\"],\"side\":\"RIGHT\"},\"type\":\"ConnectorPlacement.EquallySpacedRectSide\",\"uuid\":\"e50175c1-005c-4b0b-bced-b882197eaab2\"},{\"content\":{\"connectorIds\":[\"LConn2\"],\"side\":\"TOP\"},\"type\":\"ConnectorPlacement.EquallySpacedRectSide\",\"uuid\":\"2a04a964-d53e-47ee-8c79-d53dd599bafe\"},{\"content\":{\"connectorIds\":[\"RConn2\"],\"side\":\"BOTTOM\"},\"type\":\"ConnectorPlacement.EquallySpacedRectSide\",\"uuid\":\"a0066dd6-a193-491c-afbe-bac00dfc3505\"}]},\"type\":\"ConnectorPlacement.EquallySpacedConnector\",\"uuid\":\"c80211c6-bb24-481b-97ca-2752015f3b18\"}],\"packageUris\":[\"http://schema.mathworks.com/mf0/Connector/19700101\"],\"version\":\"1.0\"}"
  Tile51 : Subsystem  mask(Square Tile){side=side, thickness=thick, color=color2, opacity=opacity}
      mask prompts: side "Side (m) :"; thickness "Thickness (m) :"; color "Color [RGB] :"; opacity "Opacity (0...1) :"
      mask help: This block creates a flat, single, square tile element. The square tile body is mass-less, so it will not have an effect on the dynamic simulation. This square tile element can be used as a graphic reference by itself, or as part of a composite graphic reference made of an array of interconnected tiles. The square tile is aligned with the XY plane, and the block provides frame connector ports to the middle points on each of the four sides of the body of the square - right (+X), left (-X), top (+Y) and bottom (-Y). All dimensions are in meters.
      settings: PortSchema="{\"entries\":[{\"content\":{\"sides\":[{\"content\":{\"connectorIds\":[\"LConn1\"]},\"type\":\"ConnectorPlacement.EquallySpacedRectSide\",\"uuid\":\"a971723f-ea37-4e9b-910b-501b94fb0ba2\"},{\"content\":{\"connectorIds\":[\"RConn1\"],\"side\":\"RIGHT\"},\"type\":\"ConnectorPlacement.EquallySpacedRectSide\",\"uuid\":\"e50175c1-005c-4b0b-bced-b882197eaab2\"},{\"content\":{\"connectorIds\":[\"LConn2\"],\"side\":\"TOP\"},\"type\":\"ConnectorPlacement.EquallySpacedRectSide\",\"uuid\":\"2a04a964-d53e-47ee-8c79-d53dd599bafe\"},{\"content\":{\"connectorIds\":[\"RConn2\"],\"side\":\"BOTTOM\"},\"type\":\"ConnectorPlacement.EquallySpacedRectSide\",\"uuid\":\"a0066dd6-a193-491c-afbe-bac00dfc3505\"}]},\"type\":\"ConnectorPlacement.EquallySpacedConnector\",\"uuid\":\"c80211c6-bb24-481b-97ca-2752015f3b18\"}],\"packageUris\":[\"http://schema.mathworks.com/mf0/Connector/19700101\"],\"version\":\"1.0\"}"
  Tile52 : Subsystem  mask(Square Tile){side=side, thickness=thick, color=color2, opacity=opacity}
      mask prompts: side "Side (m) :"; thickness "Thickness (m) :"; color "Color [RGB] :"; opacity "Opacity (0...1) :"
      mask help: This block creates a flat, single, square tile element. The square tile body is mass-less, so it will not have an effect on the dynamic simulation. This square tile element can be used as a graphic reference by itself, or as part of a composite graphic reference made of an array of interconnected tiles. The square tile is aligned with the XY plane, and the block provides frame connector ports to the middle points on each of the four sides of the body of the square - right (+X), left (-X), top (+Y) and bottom (-Y). All dimensions are in meters.
      settings: PortSchema="{\"entries\":[{\"content\":{\"sides\":[{\"content\":{\"connectorIds\":[\"LConn1\"]},\"type\":\"ConnectorPlacement.EquallySpacedRectSide\",\"uuid\":\"a971723f-ea37-4e9b-910b-501b94fb0ba2\"},{\"content\":{\"connectorIds\":[\"RConn1\"],\"side\":\"RIGHT\"},\"type\":\"ConnectorPlacement.EquallySpacedRectSide\",\"uuid\":\"e50175c1-005c-4b0b-bced-b882197eaab2\"},{\"content\":{\"connectorIds\":[\"LConn2\"],\"side\":\"TOP\"},\"type\":\"ConnectorPlacement.EquallySpacedRectSide\",\"uuid\":\"2a04a964-d53e-47ee-8c79-d53dd599bafe\"},{\"content\":{\"connectorIds\":[\"RConn2\"],\"side\":\"BOTTOM\"},\"type\":\"ConnectorPlacement.EquallySpacedRectSide\",\"uuid\":\"a0066dd6-a193-491c-afbe-bac00dfc3505\"}]},\"type\":\"ConnectorPlacement.EquallySpacedConnector\",\"uuid\":\"c80211c6-bb24-481b-97ca-2752015f3b18\"}],\"packageUris\":[\"http://schema.mathworks.com/mf0/Connector/19700101\"],\"version\":\"1.0\"}"
  Tile53 : Subsystem  mask(Square Tile){side=side, thickness=thick, color=color1, opacity=opacity}
      mask prompts: side "Side (m) :"; thickness "Thickness (m) :"; color "Color [RGB] :"; opacity "Opacity (0...1) :"
      mask help: This block creates a flat, single, square tile element. The square tile body is mass-less, so it will not have an effect on the dynamic simulation. This square tile element can be used as a graphic reference by itself, or as part of a composite graphic reference made of an array of interconnected tiles. The square tile is aligned with the XY plane, and the block provides frame connector ports to the middle points on each of the four sides of the body of the square - right (+X), left (-X), top (+Y) and bottom (-Y). All dimensions are in meters.
      settings: PortSchema="{\"entries\":[{\"content\":{\"sides\":[{\"content\":{\"connectorIds\":[\"LConn1\"]},\"type\":\"ConnectorPlacement.EquallySpacedRectSide\",\"uuid\":\"a971723f-ea37-4e9b-910b-501b94fb0ba2\"},{\"content\":{\"connectorIds\":[\"RConn1\"],\"side\":\"RIGHT\"},\"type\":\"ConnectorPlacement.EquallySpacedRectSide\",\"uuid\":\"e50175c1-005c-4b0b-bced-b882197eaab2\"},{\"content\":{\"connectorIds\":[\"LConn2\"],\"side\":\"TOP\"},\"type\":\"ConnectorPlacement.EquallySpacedRectSide\",\"uuid\":\"2a04a964-d53e-47ee-8c79-d53dd599bafe\"},{\"content\":{\"connectorIds\":[\"RConn2\"],\"side\":\"BOTTOM\"},\"type\":\"ConnectorPlacement.EquallySpacedRectSide\",\"uuid\":\"a0066dd6-a193-491c-afbe-bac00dfc3505\"}]},\"type\":\"ConnectorPlacement.EquallySpacedConnector\",\"uuid\":\"c80211c6-bb24-481b-97ca-2752015f3b18\"}],\"packageUris\":[\"http://schema.mathworks.com/mf0/Connector/19700101\"],\"version\":\"1.0\"}"
  Tile54 : Subsystem  mask(Square Tile){side=side, thickness=thick, color=color2, opacity=opacity}
      mask prompts: side "Side (m) :"; thickness "Thickness (m) :"; color "Color [RGB] :"; opacity "Opacity (0...1) :"
      mask help: This block creates a flat, single, square tile element. The square tile body is mass-less, so it will not have an effect on the dynamic simulation. This square tile element can be used as a graphic reference by itself, or as part of a composite graphic reference made of an array of interconnected tiles. The square tile is aligned with the XY plane, and the block provides frame connector ports to the middle points on each of the four sides of the body of the square - right (+X), left (-X), top (+Y) and bottom (-Y). All dimensions are in meters.
      settings: PortSchema="{\"entries\":[{\"content\":{\"sides\":[{\"content\":{\"connectorIds\":[\"LConn1\"]},\"type\":\"ConnectorPlacement.EquallySpacedRectSide\",\"uuid\":\"a971723f-ea37-4e9b-910b-501b94fb0ba2\"},{\"content\":{\"connectorIds\":[\"RConn1\"],\"side\":\"RIGHT\"},\"type\":\"ConnectorPlacement.EquallySpacedRectSide\",\"uuid\":\"e50175c1-005c-4b0b-bced-b882197eaab2\"},{\"content\":{\"connectorIds\":[\"LConn2\"],\"side\":\"TOP\"},\"type\":\"ConnectorPlacement.EquallySpacedRectSide\",\"uuid\":\"2a04a964-d53e-47ee-8c79-d53dd599bafe\"},{\"content\":{\"connectorIds\":[\"RConn2\"],\"side\":\"BOTTOM\"},\"type\":\"ConnectorPlacement.EquallySpacedRectSide\",\"uuid\":\"a0066dd6-a193-491c-afbe-bac00dfc3505\"}]},\"type\":\"ConnectorPlacement.EquallySpacedConnector\",\"uuid\":\"c80211c6-bb24-481b-97ca-2752015f3b18\"}],\"packageUris\":[\"http://schema.mathworks.com/mf0/Connector/19700101\"],\"version\":\"1.0\"}"
  Tile55 : Subsystem  mask(Square Tile){side=side, thickness=thick, color=color1, opacity=opacity}
      mask prompts: side "Side (m) :"; thickness "Thickness (m) :"; color "Color [RGB] :"; opacity "Opacity (0...1) :"
      mask help: This block creates a flat, single, square tile element. The square tile body is mass-less, so it will not have an effect on the dynamic simulation. This square tile element can be used as a graphic reference by itself, or as part of a composite graphic reference made of an array of interconnected tiles. The square tile is aligned with the XY plane, and the block provides frame connector ports to the middle points on each of the four sides of the body of the square - right (+X), left (-X), top (+Y) and bottom (-Y). All dimensions are in meters.
      settings: PortSchema="{\"entries\":[{\"content\":{\"sides\":[{\"content\":{\"connectorIds\":[\"LConn1\"]},\"type\":\"ConnectorPlacement.EquallySpacedRectSide\",\"uuid\":\"a971723f-ea37-4e9b-910b-501b94fb0ba2\"},{\"content\":{\"connectorIds\":[\"RConn1\"],\"side\":\"RIGHT\"},\"type\":\"ConnectorPlacement.EquallySpacedRectSide\",\"uuid\":\"e50175c1-005c-4b0b-bced-b882197eaab2\"},{\"content\":{\"connectorIds\":[\"LConn2\"],\"side\":\"TOP\"},\"type\":\"ConnectorPlacement.EquallySpacedRectSide\",\"uuid\":\"2a04a964-d53e-47ee-8c79-d53dd599bafe\"},{\"content\":{\"connectorIds\":[\"RConn2\"],\"side\":\"BOTTOM\"},\"type\":\"ConnectorPlacement.EquallySpacedRectSide\",\"uuid\":\"a0066dd6-a193-491c-afbe-bac00dfc3505\"}]},\"type\":\"ConnectorPlacement.EquallySpacedConnector\",\"uuid\":\"c80211c6-bb24-481b-97ca-2752015f3b18\"}],\"packageUris\":[\"http://schema.mathworks.com/mf0/Connector/19700101\"],\"version\":\"1.0\"}"
  Tile56 : Subsystem  mask(Square Tile){side=side, thickness=thick, color=color2, opacity=opacity}
      mask prompts: side "Side (m) :"; thickness "Thickness (m) :"; color "Color [RGB] :"; opacity "Opacity (0...1) :"
      mask help: This block creates a flat, single, square tile element. The square tile body is mass-less, so it will not have an effect on the dynamic simulation. This square tile element can be used as a graphic reference by itself, or as part of a composite graphic reference made of an array of interconnected tiles. The square tile is aligned with the XY plane, and the block provides frame connector ports to the middle points on each of the four sides of the body of the square - right (+X), left (-X), top (+Y) and bottom (-Y). All dimensions are in meters.
      settings: PortSchema="{\"entries\":[{\"content\":{\"sides\":[{\"content\":{\"connectorIds\":[\"LConn1\"]},\"type\":\"ConnectorPlacement.EquallySpacedRectSide\",\"uuid\":\"a971723f-ea37-4e9b-910b-501b94fb0ba2\"},{\"content\":{\"connectorIds\":[\"RConn1\"],\"side\":\"RIGHT\"},\"type\":\"ConnectorPlacement.EquallySpacedRectSide\",\"uuid\":\"e50175c1-005c-4b0b-bced-b882197eaab2\"},{\"content\":{\"connectorIds\":[\"LConn2\"],\"side\":\"TOP\"},\"type\":\"ConnectorPlacement.EquallySpacedRectSide\",\"uuid\":\"2a04a964-d53e-47ee-8c79-d53dd599bafe\"},{\"content\":{\"connectorIds\":[\"RConn2\"],\"side\":\"BOTTOM\"},\"type\":\"ConnectorPlacement.EquallySpacedRectSide\",\"uuid\":\"a0066dd6-a193-491c-afbe-bac00dfc3505\"}]},\"type\":\"ConnectorPlacement.EquallySpacedConnector\",\"uuid\":\"c80211c6-bb24-481b-97ca-2752015f3b18\"}],\"packageUris\":[\"http://schema.mathworks.com/mf0/Connector/19700101\"],\"version\":\"1.0\"}"
  Tile57 : Subsystem  mask(Square Tile){side=side, thickness=thick, color=color1, opacity=opacity}
      mask prompts: side "Side (m) :"; thickness "Thickness (m) :"; color "Color [RGB] :"; opacity "Opacity (0...1) :"
      mask help: This block creates a flat, single, square tile element. The square tile body is mass-less, so it will not have an effect on the dynamic simulation. This square tile element can be used as a graphic reference by itself, or as part of a composite graphic reference made of an array of interconnected tiles. The square tile is aligned with the XY plane, and the block provides frame connector ports to the middle points on each of the four sides of the body of the square - right (+X), left (-X), top (+Y) and bottom (-Y). All dimensions are in meters.
      settings: PortSchema="{\"entries\":[{\"content\":{\"sides\":[{\"content\":{\"connectorIds\":[\"LConn1\"]},\"type\":\"ConnectorPlacement.EquallySpacedRectSide\",\"uuid\":\"a971723f-ea37-4e9b-910b-501b94fb0ba2\"},{\"content\":{\"connectorIds\":[\"RConn1\"],\"side\":\"RIGHT\"},\"type\":\"ConnectorPlacement.EquallySpacedRectSide\",\"uuid\":\"e50175c1-005c-4b0b-bced-b882197eaab2\"},{\"content\":{\"connectorIds\":[\"LConn2\"],\"side\":\"TOP\"},\"type\":\"ConnectorPlacement.EquallySpacedRectSide\",\"uuid\":\"2a04a964-d53e-47ee-8c79-d53dd599bafe\"},{\"content\":{\"connectorIds\":[\"RConn2\"],\"side\":\"BOTTOM\"},\"type\":\"ConnectorPlacement.EquallySpacedRectSide\",\"uuid\":\"a0066dd6-a193-491c-afbe-bac00dfc3505\"}]},\"type\":\"ConnectorPlacement.EquallySpacedConnector\",\"uuid\":\"c80211c6-bb24-481b-97ca-2752015f3b18\"}],\"packageUris\":[\"http://schema.mathworks.com/mf0/Connector/19700101\"],\"version\":\"1.0\"}"
  Tile58 : Subsystem  mask(Square Tile){side=side, thickness=thick, color=color2, opacity=opacity}
      mask prompts: side "Side (m) :"; thickness "Thickness (m) :"; color "Color [RGB] :"; opacity "Opacity (0...1) :"
      mask help: This block creates a flat, single, square tile element. The square tile body is mass-less, so it will not have an effect on the dynamic simulation. This square tile element can be used as a graphic reference by itself, or as part of a composite graphic reference made of an array of interconnected tiles. The square tile is aligned with the XY plane, and the block provides frame connector ports to the middle points on each of the four sides of the body of the square - right (+X), left (-X), top (+Y) and bottom (-Y). All dimensions are in meters.
      settings: PortSchema="{\"entries\":[{\"content\":{\"sides\":[{\"content\":{\"connectorIds\":[\"LConn1\"]},\"type\":\"ConnectorPlacement.EquallySpacedRectSide\",\"uuid\":\"a971723f-ea37-4e9b-910b-501b94fb0ba2\"},{\"content\":{\"connectorIds\":[\"RConn1\"],\"side\":\"RIGHT\"},\"type\":\"ConnectorPlacement.EquallySpacedRectSide\",\"uuid\":\"e50175c1-005c-4b0b-bced-b882197eaab2\"},{\"content\":{\"connectorIds\":[\"LConn2\"],\"side\":\"TOP\"},\"type\":\"ConnectorPlacement.EquallySpacedRectSide\",\"uuid\":\"2a04a964-d53e-47ee-8c79-d53dd599bafe\"},{\"content\":{\"connectorIds\":[\"RConn2\"],\"side\":\"BOTTOM\"},\"type\":\"ConnectorPlacement.EquallySpacedRectSide\",\"uuid\":\"a0066dd6-a193-491c-afbe-bac00dfc3505\"}]},\"type\":\"ConnectorPlacement.EquallySpacedConnector\",\"uuid\":\"c80211c6-bb24-481b-97ca-2752015f3b18\"}],\"packageUris\":[\"http://schema.mathworks.com/mf0/Connector/19700101\"],\"version\":\"1.0\"}"
  Tile59 : Subsystem  mask(Square Tile){side=side, thickness=thick, color=color1, opacity=opacity}
      mask prompts: side "Side (m) :"; thickness "Thickness (m) :"; color "Color [RGB] :"; opacity "Opacity (0...1) :"
      mask help: This block creates a flat, single, square tile element. The square tile body is mass-less, so it will not have an effect on the dynamic simulation. This square tile element can be used as a graphic reference by itself, or as part of a composite graphic reference made of an array of interconnected tiles. The square tile is aligned with the XY plane, and the block provides frame connector ports to the middle points on each of the four sides of the body of the square - right (+X), left (-X), top (+Y) and bottom (-Y). All dimensions are in meters.
      settings: PortSchema="{\"entries\":[{\"content\":{\"sides\":[{\"content\":{\"connectorIds\":[\"LConn1\"]},\"type\":\"ConnectorPlacement.EquallySpacedRectSide\",\"uuid\":\"a971723f-ea37-4e9b-910b-501b94fb0ba2\"},{\"content\":{\"connectorIds\":[\"RConn1\"],\"side\":\"RIGHT\"},\"type\":\"ConnectorPlacement.EquallySpacedRectSide\",\"uuid\":\"e50175c1-005c-4b0b-bced-b882197eaab2\"},{\"content\":{\"connectorIds\":[\"LConn2\"],\"side\":\"TOP\"},\"type\":\"ConnectorPlacement.EquallySpacedRectSide\",\"uuid\":\"2a04a964-d53e-47ee-8c79-d53dd599bafe\"},{\"content\":{\"connectorIds\":[\"RConn2\"],\"side\":\"BOTTOM\"},\"type\":\"ConnectorPlacement.EquallySpacedRectSide\",\"uuid\":\"a0066dd6-a193-491c-afbe-bac00dfc3505\"}]},\"type\":\"ConnectorPlacement.EquallySpacedConnector\",\"uuid\":\"c80211c6-bb24-481b-97ca-2752015f3b18\"}],\"packageUris\":[\"http://schema.mathworks.com/mf0/Connector/19700101\"],\"version\":\"1.0\"}"
  Tile6 : Subsystem  mask(Square Tile){side=side, thickness=thick, color=color2, opacity=opacity}
      mask prompts: side "Side (m) :"; thickness "Thickness (m) :"; color "Color [RGB] :"; opacity "Opacity (0...1) :"
      mask help: This block creates a flat, single, square tile element. The square tile body is mass-less, so it will not have an effect on the dynamic simulation. This square tile element can be used as a graphic reference by itself, or as part of a composite graphic reference made of an array of interconnected tiles. The square tile is aligned with the XY plane, and the block provides frame connector ports to the middle points on each of the four sides of the body of the square - right (+X), left (-X), top (+Y) and bottom (-Y). All dimensions are in meters.
      settings: PortSchema="{\"entries\":[{\"content\":{\"sides\":[{\"content\":{\"connectorIds\":[\"LConn1\"]},\"type\":\"ConnectorPlacement.EquallySpacedRectSide\",\"uuid\":\"a971723f-ea37-4e9b-910b-501b94fb0ba2\"},{\"content\":{\"connectorIds\":[\"RConn1\"],\"side\":\"RIGHT\"},\"type\":\"ConnectorPlacement.EquallySpacedRectSide\",\"uuid\":\"e50175c1-005c-4b0b-bced-b882197eaab2\"},{\"content\":{\"connectorIds\":[\"LConn2\"],\"side\":\"TOP\"},\"type\":\"ConnectorPlacement.EquallySpacedRectSide\",\"uuid\":\"2a04a964-d53e-47ee-8c79-d53dd599bafe\"},{\"content\":{\"connectorIds\":[\"RConn2\"],\"side\":\"BOTTOM\"},\"type\":\"ConnectorPlacement.EquallySpacedRectSide\",\"uuid\":\"a0066dd6-a193-491c-afbe-bac00dfc3505\"}]},\"type\":\"ConnectorPlacement.EquallySpacedConnector\",\"uuid\":\"c80211c6-bb24-481b-97ca-2752015f3b18\"}],\"packageUris\":[\"http://schema.mathworks.com/mf0/Connector/19700101\"],\"version\":\"1.0\"}"
  Tile60 : Subsystem  mask(Square Tile){side=side, thickness=thick, color=color1, opacity=opacity}
      mask prompts: side "Side (m) :"; thickness "Thickness (m) :"; color "Color [RGB] :"; opacity "Opacity (0...1) :"
      mask help: This block creates a flat, single, square tile element. The square tile body is mass-less, so it will not have an effect on the dynamic simulation. This square tile element can be used as a graphic reference by itself, or as part of a composite graphic reference made of an array of interconnected tiles. The square tile is aligned with the XY plane, and the block provides frame connector ports to the middle points on each of the four sides of the body of the square - right (+X), left (-X), top (+Y) and bottom (-Y). All dimensions are in meters.
      settings: PortSchema="{\"entries\":[{\"content\":{\"sides\":[{\"content\":{\"connectorIds\":[\"LConn1\"]},\"type\":\"ConnectorPlacement.EquallySpacedRectSide\",\"uuid\":\"a971723f-ea37-4e9b-910b-501b94fb0ba2\"},{\"content\":{\"connectorIds\":[\"RConn1\"],\"side\":\"RIGHT\"},\"type\":\"ConnectorPlacement.EquallySpacedRectSide\",\"uuid\":\"e50175c1-005c-4b0b-bced-b882197eaab2\"},{\"content\":{\"connectorIds\":[\"LConn2\"],\"side\":\"TOP\"},\"type\":\"ConnectorPlacement.EquallySpacedRectSide\",\"uuid\":\"2a04a964-d53e-47ee-8c79-d53dd599bafe\"},{\"content\":{\"connectorIds\":[\"RConn2\"],\"side\":\"BOTTOM\"},\"type\":\"ConnectorPlacement.EquallySpacedRectSide\",\"uuid\":\"a0066dd6-a193-491c-afbe-bac00dfc3505\"}]},\"type\":\"ConnectorPlacement.EquallySpacedConnector\",\"uuid\":\"c80211c6-bb24-481b-97ca-2752015f3b18\"}],\"packageUris\":[\"http://schema.mathworks.com/mf0/Connector/19700101\"],\"version\":\"1.0\"}"
  Tile7 : Subsystem  mask(Square Tile){side=side, thickness=thick, color=color1, opacity=opacity}
      mask prompts: side "Side (m) :"; thickness "Thickness (m) :"; color "Color [RGB] :"; opacity "Opacity (0...1) :"
      mask help: This block creates a flat, single, square tile element. The square tile body is mass-less, so it will not have an effect on the dynamic simulation. This square tile element can be used as a graphic reference by itself, or as part of a composite graphic reference made of an array of interconnected tiles. The square tile is aligned with the XY plane, and the block provides frame connector ports to the middle points on each of the four sides of the body of the square - right (+X), left (-X), top (+Y) and bottom (-Y). All dimensions are in meters.
      settings: PortSchema="{\"entries\":[{\"content\":{\"sides\":[{\"content\":{\"connectorIds\":[\"LConn1\"]},\"type\":\"ConnectorPlacement.EquallySpacedRectSide\",\"uuid\":\"a971723f-ea37-4e9b-910b-501b94fb0ba2\"},{\"content\":{\"connectorIds\":[\"RConn1\"],\"side\":\"RIGHT\"},\"type\":\"ConnectorPlacement.EquallySpacedRectSide\",\"uuid\":\"e50175c1-005c-4b0b-bced-b882197eaab2\"},{\"content\":{\"connectorIds\":[\"LConn2\"],\"side\":\"TOP\"},\"type\":\"ConnectorPlacement.EquallySpacedRectSide\",\"uuid\":\"2a04a964-d53e-47ee-8c79-d53dd599bafe\"},{\"content\":{\"connectorIds\":[\"RConn2\"],\"side\":\"BOTTOM\"},\"type\":\"ConnectorPlacement.EquallySpacedRectSide\",\"uuid\":\"a0066dd6-a193-491c-afbe-bac00dfc3505\"}]},\"type\":\"ConnectorPlacement.EquallySpacedConnector\",\"uuid\":\"c80211c6-bb24-481b-97ca-2752015f3b18\"}],\"packageUris\":[\"http://schema.mathworks.com/mf0/Connector/19700101\"],\"version\":\"1.0\"}"
  Tile71 : Subsystem  mask(Square Tile){side=side, thickness=thick, color=color1, opacity=opacity}
      mask prompts: side "Side (m) :"; thickness "Thickness (m) :"; color "Color [RGB] :"; opacity "Opacity (0...1) :"
      mask help: This block creates a flat, single, square tile element. The square tile body is mass-less, so it will not have an effect on the dynamic simulation. This square tile element can be used as a graphic reference by itself, or as part of a composite graphic reference made of an array of interconnected tiles. The square tile is aligned with the XY plane, and the block provides frame connector ports to the middle points on each of the four sides of the body of the square - right (+X), left (-X), top (+Y) and bottom (-Y). All dimensions are in meters.
      settings: PortSchema="{\"entries\":[{\"content\":{\"sides\":[{\"content\":{\"connectorIds\":[\"LConn1\"]},\"type\":\"ConnectorPlacement.EquallySpacedRectSide\",\"uuid\":\"a971723f-ea37-4e9b-910b-501b94fb0ba2\"},{\"content\":{\"connectorIds\":[\"RConn1\"],\"side\":\"RIGHT\"},\"type\":\"ConnectorPlacement.EquallySpacedRectSide\",\"uuid\":\"e50175c1-005c-4b0b-bced-b882197eaab2\"},{\"content\":{\"connectorIds\":[\"LConn2\"],\"side\":\"TOP\"},\"type\":\"ConnectorPlacement.EquallySpacedRectSide\",\"uuid\":\"2a04a964-d53e-47ee-8c79-d53dd599bafe\"},{\"content\":{\"connectorIds\":[\"RConn2\"],\"side\":\"BOTTOM\"},\"type\":\"ConnectorPlacement.EquallySpacedRectSide\",\"uuid\":\"a0066dd6-a193-491c-afbe-bac00dfc3505\"}]},\"type\":\"ConnectorPlacement.EquallySpacedConnector\",\"uuid\":\"c80211c6-bb24-481b-97ca-2752015f3b18\"}],\"packageUris\":[\"http://schema.mathworks.com/mf0/Connector/19700101\"],\"version\":\"1.0\"}"
  Tile72 : Subsystem  mask(Square Tile){side=side, thickness=thick, color=color2, opacity=opacity}
      mask prompts: side "Side (m) :"; thickness "Thickness (m) :"; color "Color [RGB] :"; opacity "Opacity (0...1) :"
      mask help: This block creates a flat, single, square tile element. The square tile body is mass-less, so it will not have an effect on the dynamic simulation. This square tile element can be used as a graphic reference by itself, or as part of a composite graphic reference made of an array of interconnected tiles. The square tile is aligned with the XY plane, and the block provides frame connector ports to the middle points on each of the four sides of the body of the square - right (+X), left (-X), top (+Y) and bottom (-Y). All dimensions are in meters.
      settings: PortSchema="{\"entries\":[{\"content\":{\"sides\":[{\"content\":{\"connectorIds\":[\"LConn1\"]},\"type\":\"ConnectorPlacement.EquallySpacedRectSide\",\"uuid\":\"a971723f-ea37-4e9b-910b-501b94fb0ba2\"},{\"content\":{\"connectorIds\":[\"RConn1\"],\"side\":\"RIGHT\"},\"type\":\"ConnectorPlacement.EquallySpacedRectSide\",\"uuid\":\"e50175c1-005c-4b0b-bced-b882197eaab2\"},{\"content\":{\"connectorIds\":[\"LConn2\"],\"side\":\"TOP\"},\"type\":\"ConnectorPlacement.EquallySpacedRectSide\",\"uuid\":\"2a04a964-d53e-47ee-8c79-d53dd599bafe\"},{\"content\":{\"connectorIds\":[\"RConn2\"],\"side\":\"BOTTOM\"},\"type\":\"ConnectorPlacement.EquallySpacedRectSide\",\"uuid\":\"a0066dd6-a193-491c-afbe-bac00dfc3505\"}]},\"type\":\"ConnectorPlacement.EquallySpacedConnector\",\"uuid\":\"c80211c6-bb24-481b-97ca-2752015f3b18\"}],\"packageUris\":[\"http://schema.mathworks.com/mf0/Connector/19700101\"],\"version\":\"1.0\"}"
  Tile73 : Subsystem  mask(Square Tile){side=side, thickness=thick, color=color2, opacity=opacity}
      mask prompts: side "Side (m) :"; thickness "Thickness (m) :"; color "Color [RGB] :"; opacity "Opacity (0...1) :"
      mask help: This block creates a flat, single, square tile element. The square tile body is mass-less, so it will not have an effect on the dynamic simulation. This square tile element can be used as a graphic reference by itself, or as part of a composite graphic reference made of an array of interconnected tiles. The square tile is aligned with the XY plane, and the block provides frame connector ports to the middle points on each of the four sides of the body of the square - right (+X), left (-X), top (+Y) and bottom (-Y). All dimensions are in meters.
      settings: PortSchema="{\"entries\":[{\"content\":{\"sides\":[{\"content\":{\"connectorIds\":[\"LConn1\"]},\"type\":\"ConnectorPlacement.EquallySpacedRectSide\",\"uuid\":\"a971723f-ea37-4e9b-910b-501b94fb0ba2\"},{\"content\":{\"connectorIds\":[\"RConn1\"],\"side\":\"RIGHT\"},\"type\":\"ConnectorPlacement.EquallySpacedRectSide\",\"uuid\":\"e50175c1-005c-4b0b-bced-b882197eaab2\"},{\"content\":{\"connectorIds\":[\"LConn2\"],\"side\":\"TOP\"},\"type\":\"ConnectorPlacement.EquallySpacedRectSide\",\"uuid\":\"2a04a964-d53e-47ee-8c79-d53dd599bafe\"},{\"content\":{\"connectorIds\":[\"RConn2\"],\"side\":\"BOTTOM\"},\"type\":\"ConnectorPlacement.EquallySpacedRectSide\",\"uuid\":\"a0066dd6-a193-491c-afbe-bac00dfc3505\"}]},\"type\":\"ConnectorPlacement.EquallySpacedConnector\",\"uuid\":\"c80211c6-bb24-481b-97ca-2752015f3b18\"}],\"packageUris\":[\"http://schema.mathworks.com/mf0/Connector/19700101\"],\"version\":\"1.0\"}"
  Tile74 : Subsystem  mask(Square Tile){side=side, thickness=thick, color=color2, opacity=opacity}
      mask prompts: side "Side (m) :"; thickness "Thickness (m) :"; color "Color [RGB] :"; opacity "Opacity (0...1) :"
      mask help: This block creates a flat, single, square tile element. The square tile body is mass-less, so it will not have an effect on the dynamic simulation. This square tile element can be used as a graphic reference by itself, or as part of a composite graphic reference made of an array of interconnected tiles. The square tile is aligned with the XY plane, and the block provides frame connector ports to the middle points on each of the four sides of the body of the square - right (+X), left (-X), top (+Y) and bottom (-Y). All dimensions are in meters.
      settings: PortSchema="{\"entries\":[{\"content\":{\"sides\":[{\"content\":{\"connectorIds\":[\"LConn1\"]},\"type\":\"ConnectorPlacement.EquallySpacedRectSide\",\"uuid\":\"a971723f-ea37-4e9b-910b-501b94fb0ba2\"},{\"content\":{\"connectorIds\":[\"RConn1\"],\"side\":\"RIGHT\"},\"type\":\"ConnectorPlacement.EquallySpacedRectSide\",\"uuid\":\"e50175c1-005c-4b0b-bced-b882197eaab2\"},{\"content\":{\"connectorIds\":[\"LConn2\"],\"side\":\"TOP\"},\"type\":\"ConnectorPlacement.EquallySpacedRectSide\",\"uuid\":\"2a04a964-d53e-47ee-8c79-d53dd599bafe\"},{\"content\":{\"connectorIds\":[\"RConn2\"],\"side\":\"BOTTOM\"},\"type\":\"ConnectorPlacement.EquallySpacedRectSide\",\"uuid\":\"a0066dd6-a193-491c-afbe-bac00dfc3505\"}]},\"type\":\"ConnectorPlacement.EquallySpacedConnector\",\"uuid\":\"c80211c6-bb24-481b-97ca-2752015f3b18\"}],\"packageUris\":[\"http://schema.mathworks.com/mf0/Connector/19700101\"],\"version\":\"1.0\"}"
  Tile75 : Subsystem  mask(Square Tile){side=side, thickness=thick, color=color1, opacity=opacity}
      mask prompts: side "Side (m) :"; thickness "Thickness (m) :"; color "Color [RGB] :"; opacity "Opacity (0...1) :"
      mask help: This block creates a flat, single, square tile element. The square tile body is mass-less, so it will not have an effect on the dynamic simulation. This square tile element can be used as a graphic reference by itself, or as part of a composite graphic reference made of an array of interconnected tiles. The square tile is aligned with the XY plane, and the block provides frame connector ports to the middle points on each of the four sides of the body of the square - right (+X), left (-X), top (+Y) and bottom (-Y). All dimensions are in meters.
      settings: PortSchema="{\"entries\":[{\"content\":{\"sides\":[{\"content\":{\"connectorIds\":[\"LConn1\"]},\"type\":\"ConnectorPlacement.EquallySpacedRectSide\",\"uuid\":\"a971723f-ea37-4e9b-910b-501b94fb0ba2\"},{\"content\":{\"connectorIds\":[\"RConn1\"],\"side\":\"RIGHT\"},\"type\":\"ConnectorPlacement.EquallySpacedRectSide\",\"uuid\":\"e50175c1-005c-4b0b-bced-b882197eaab2\"},{\"content\":{\"connectorIds\":[\"LConn2\"],\"side\":\"TOP\"},\"type\":\"ConnectorPlacement.EquallySpacedRectSide\",\"uuid\":\"2a04a964-d53e-47ee-8c79-d53dd599bafe\"},{\"content\":{\"connectorIds\":[\"RConn2\"],\"side\":\"BOTTOM\"},\"type\":\"ConnectorPlacement.EquallySpacedRectSide\",\"uuid\":\"a0066dd6-a193-491c-afbe-bac00dfc3505\"}]},\"type\":\"ConnectorPlacement.EquallySpacedConnector\",\"uuid\":\"c80211c6-bb24-481b-97ca-2752015f3b18\"}],\"packageUris\":[\"http://schema.mathworks.com/mf0/Connector/19700101\"],\"version\":\"1.0\"}"
  Tile76 : Subsystem  mask(Square Tile){side=side, thickness=thick, color=color2, opacity=opacity}
      mask prompts: side "Side (m) :"; thickness "Thickness (m) :"; color "Color [RGB] :"; opacity "Opacity (0...1) :"
      mask help: This block creates a flat, single, square tile element. The square tile body is mass-less, so it will not have an effect on the dynamic simulation. This square tile element can be used as a graphic reference by itself, or as part of a composite graphic reference made of an array of interconnected tiles. The square tile is aligned with the XY plane, and the block provides frame connector ports to the middle points on each of the four sides of the body of the square - right (+X), left (-X), top (+Y) and bottom (-Y). All dimensions are in meters.
      settings: PortSchema="{\"entries\":[{\"content\":{\"sides\":[{\"content\":{\"connectorIds\":[\"LConn1\"]},\"type\":\"ConnectorPlacement.EquallySpacedRectSide\",\"uuid\":\"a971723f-ea37-4e9b-910b-501b94fb0ba2\"},{\"content\":{\"connectorIds\":[\"RConn1\"],\"side\":\"RIGHT\"},\"type\":\"ConnectorPlacement.EquallySpacedRectSide\",\"uuid\":\"e50175c1-005c-4b0b-bced-b882197eaab2\"},{\"content\":{\"connectorIds\":[\"LConn2\"],\"side\":\"TOP\"},\"type\":\"ConnectorPlacement.EquallySpacedRectSide\",\"uuid\":\"2a04a964-d53e-47ee-8c79-d53dd599bafe\"},{\"content\":{\"connectorIds\":[\"RConn2\"],\"side\":\"BOTTOM\"},\"type\":\"ConnectorPlacement.EquallySpacedRectSide\",\"uuid\":\"a0066dd6-a193-491c-afbe-bac00dfc3505\"}]},\"type\":\"ConnectorPlacement.EquallySpacedConnector\",\"uuid\":\"c80211c6-bb24-481b-97ca-2752015f3b18\"}],\"packageUris\":[\"http://schema.mathworks.com/mf0/Connector/19700101\"],\"version\":\"1.0\"}"
  Tile77 : Subsystem  mask(Square Tile){side=side, thickness=thick, color=color1, opacity=opacity}
      mask prompts: side "Side (m) :"; thickness "Thickness (m) :"; color "Color [RGB] :"; opacity "Opacity (0...1) :"
      mask help: This block creates a flat, single, square tile element. The square tile body is mass-less, so it will not have an effect on the dynamic simulation. This square tile element can be used as a graphic reference by itself, or as part of a composite graphic reference made of an array of interconnected tiles. The square tile is aligned with the XY plane, and the block provides frame connector ports to the middle points on each of the four sides of the body of the square - right (+X), left (-X), top (+Y) and bottom (-Y). All dimensions are in meters.
      settings: PortSchema="{\"entries\":[{\"content\":{\"sides\":[{\"content\":{\"connectorIds\":[\"LConn1\"]},\"type\":\"ConnectorPlacement.EquallySpacedRectSide\",\"uuid\":\"a971723f-ea37-4e9b-910b-501b94fb0ba2\"},{\"content\":{\"connectorIds\":[\"RConn1\"],\"side\":\"RIGHT\"},\"type\":\"ConnectorPlacement.EquallySpacedRectSide\",\"uuid\":\"e50175c1-005c-4b0b-bced-b882197eaab2\"},{\"content\":{\"connectorIds\":[\"LConn2\"],\"side\":\"TOP\"},\"type\":\"ConnectorPlacement.EquallySpacedRectSide\",\"uuid\":\"2a04a964-d53e-47ee-8c79-d53dd599bafe\"},{\"content\":{\"connectorIds\":[\"RConn2\"],\"side\":\"BOTTOM\"},\"type\":\"ConnectorPlacement.EquallySpacedRectSide\",\"uuid\":\"a0066dd6-a193-491c-afbe-bac00dfc3505\"}]},\"type\":\"ConnectorPlacement.EquallySpacedConnector\",\"uuid\":\"c80211c6-bb24-481b-97ca-2752015f3b18\"}],\"packageUris\":[\"http://schema.mathworks.com/mf0/Connector/19700101\"],\"version\":\"1.0\"}"
  Tile78 : Subsystem  mask(Square Tile){side=side, thickness=thick, color=color2, opacity=opacity}
      mask prompts: side "Side (m) :"; thickness "Thickness (m) :"; color "Color [RGB] :"; opacity "Opacity (0...1) :"
      mask help: This block creates a flat, single, square tile element. The square tile body is mass-less, so it will not have an effect on the dynamic simulation. This square tile element can be used as a graphic reference by itself, or as part of a composite graphic reference made of an array of interconnected tiles. The square tile is aligned with the XY plane, and the block provides frame connector ports to the middle points on each of the four sides of the body of the square - right (+X), left (-X), top (+Y) and bottom (-Y). All dimensions are in meters.
      settings: PortSchema="{\"entries\":[{\"content\":{\"sides\":[{\"content\":{\"connectorIds\":[\"LConn1\"]},\"type\":\"ConnectorPlacement.EquallySpacedRectSide\",\"uuid\":\"a971723f-ea37-4e9b-910b-501b94fb0ba2\"},{\"content\":{\"connectorIds\":[\"RConn1\"],\"side\":\"RIGHT\"},\"type\":\"ConnectorPlacement.EquallySpacedRectSide\",\"uuid\":\"e50175c1-005c-4b0b-bced-b882197eaab2\"},{\"content\":{\"connectorIds\":[\"LConn2\"],\"side\":\"TOP\"},\"type\":\"ConnectorPlacement.EquallySpacedRectSide\",\"uuid\":\"2a04a964-d53e-47ee-8c79-d53dd599bafe\"},{\"content\":{\"connectorIds\":[\"RConn2\"],\"side\":\"BOTTOM\"},\"type\":\"ConnectorPlacement.EquallySpacedRectSide\",\"uuid\":\"a0066dd6-a193-491c-afbe-bac00dfc3505\"}]},\"type\":\"ConnectorPlacement.EquallySpacedConnector\",\"uuid\":\"c80211c6-bb24-481b-97ca-2752015f3b18\"}],\"packageUris\":[\"http://schema.mathworks.com/mf0/Connector/19700101\"],\"version\":\"1.0\"}"
  Tile79 : Subsystem  mask(Square Tile){side=side, thickness=thick, color=color1, opacity=opacity}
      mask prompts: side "Side (m) :"; thickness "Thickness (m) :"; color "Color [RGB] :"; opacity "Opacity (0...1) :"
      mask help: This block creates a flat, single, square tile element. The square tile body is mass-less, so it will not have an effect on the dynamic simulation. This square tile element can be used as a graphic reference by itself, or as part of a composite graphic reference made of an array of interconnected tiles. The square tile is aligned with the XY plane, and the block provides frame connector ports to the middle points on each of the four sides of the body of the square - right (+X), left (-X), top (+Y) and bottom (-Y). All dimensions are in meters.
      settings: PortSchema="{\"entries\":[{\"content\":{\"sides\":[{\"content\":{\"connectorIds\":[\"LConn1\"]},\"type\":\"ConnectorPlacement.EquallySpacedRectSide\",\"uuid\":\"a971723f-ea37-4e9b-910b-501b94fb0ba2\"},{\"content\":{\"connectorIds\":[\"RConn1\"],\"side\":\"RIGHT\"},\"type\":\"ConnectorPlacement.EquallySpacedRectSide\",\"uuid\":\"e50175c1-005c-4b0b-bced-b882197eaab2\"},{\"content\":{\"connectorIds\":[\"LConn2\"],\"side\":\"TOP\"},\"type\":\"ConnectorPlacement.EquallySpacedRectSide\",\"uuid\":\"2a04a964-d53e-47ee-8c79-d53dd599bafe\"},{\"content\":{\"connectorIds\":[\"RConn2\"],\"side\":\"BOTTOM\"},\"type\":\"ConnectorPlacement.EquallySpacedRectSide\",\"uuid\":\"a0066dd6-a193-491c-afbe-bac00dfc3505\"}]},\"type\":\"ConnectorPlacement.EquallySpacedConnector\",\"uuid\":\"c80211c6-bb24-481b-97ca-2752015f3b18\"}],\"packageUris\":[\"http://schema.mathworks.com/mf0/Connector/19700101\"],\"version\":\"1.0\"}"
  Tile8 : Subsystem  mask(Square Tile){side=side, thickness=thick, color=color2, opacity=opacity}
      mask prompts: side "Side (m) :"; thickness "Thickness (m) :"; color "Color [RGB] :"; opacity "Opacity (0...1) :"
      mask help: This block creates a flat, single, square tile element. The square tile body is mass-less, so it will not have an effect on the dynamic simulation. This square tile element can be used as a graphic reference by itself, or as part of a composite graphic reference made of an array of interconnected tiles. The square tile is aligned with the XY plane, and the block provides frame connector ports to the middle points on each of the four sides of the body of the square - right (+X), left (-X), top (+Y) and bottom (-Y). All dimensions are in meters.
      settings: PortSchema="{\"entries\":[{\"content\":{\"sides\":[{\"content\":{\"connectorIds\":[\"LConn1\"]},\"type\":\"ConnectorPlacement.EquallySpacedRectSide\",\"uuid\":\"a971723f-ea37-4e9b-910b-501b94fb0ba2\"},{\"content\":{\"connectorIds\":[\"RConn1\"],\"side\":\"RIGHT\"},\"type\":\"ConnectorPlacement.EquallySpacedRectSide\",\"uuid\":\"e50175c1-005c-4b0b-bced-b882197eaab2\"},{\"content\":{\"connectorIds\":[\"LConn2\"],\"side\":\"TOP\"},\"type\":\"ConnectorPlacement.EquallySpacedRectSide\",\"uuid\":\"2a04a964-d53e-47ee-8c79-d53dd599bafe\"},{\"content\":{\"connectorIds\":[\"RConn2\"],\"side\":\"BOTTOM\"},\"type\":\"ConnectorPlacement.EquallySpacedRectSide\",\"uuid\":\"a0066dd6-a193-491c-afbe-bac00dfc3505\"}]},\"type\":\"ConnectorPlacement.EquallySpacedConnector\",\"uuid\":\"c80211c6-bb24-481b-97ca-2752015f3b18\"}],\"packageUris\":[\"http://schema.mathworks.com/mf0/Connector/19700101\"],\"version\":\"1.0\"}"
  Tile80 : Subsystem  mask(Square Tile){side=side, thickness=thick, color=color2, opacity=opacity}
      mask prompts: side "Side (m) :"; thickness "Thickness (m) :"; color "Color [RGB] :"; opacity "Opacity (0...1) :"
      mask help: This block creates a flat, single, square tile element. The square tile body is mass-less, so it will not have an effect on the dynamic simulation. This square tile element can be used as a graphic reference by itself, or as part of a composite graphic reference made of an array of interconnected tiles. The square tile is aligned with the XY plane, and the block provides frame connector ports to the middle points on each of the four sides of the body of the square - right (+X), left (-X), top (+Y) and bottom (-Y). All dimensions are in meters.
      settings: PortSchema="{\"entries\":[{\"content\":{\"sides\":[{\"content\":{\"connectorIds\":[\"LConn1\"]},\"type\":\"ConnectorPlacement.EquallySpacedRectSide\",\"uuid\":\"a971723f-ea37-4e9b-910b-501b94fb0ba2\"},{\"content\":{\"connectorIds\":[\"RConn1\"],\"side\":\"RIGHT\"},\"type\":\"ConnectorPlacement.EquallySpacedRectSide\",\"uuid\":\"e50175c1-005c-4b0b-bced-b882197eaab2\"},{\"content\":{\"connectorIds\":[\"LConn2\"],\"side\":\"TOP\"},\"type\":\"ConnectorPlacement.EquallySpacedRectSide\",\"uuid\":\"2a04a964-d53e-47ee-8c79-d53dd599bafe\"},{\"content\":{\"connectorIds\":[\"RConn2\"],\"side\":\"BOTTOM\"},\"type\":\"ConnectorPlacement.EquallySpacedRectSide\",\"uuid\":\"a0066dd6-a193-491c-afbe-bac00dfc3505\"}]},\"type\":\"ConnectorPlacement.EquallySpacedConnector\",\"uuid\":\"c80211c6-bb24-481b-97ca-2752015f3b18\"}],\"packageUris\":[\"http://schema.mathworks.com/mf0/Connector/19700101\"],\"version\":\"1.0\"}"
  Tile81 : Subsystem  mask(Square Tile){side=side, thickness=thick, color=color1, opacity=opacity}
      mask prompts: side "Side (m) :"; thickness "Thickness (m) :"; color "Color [RGB] :"; opacity "Opacity (0...1) :"
      mask help: This block creates a flat, single, square tile element. The square tile body is mass-less, so it will not have an effect on the dynamic simulation. This square tile element can be used as a graphic reference by itself, or as part of a composite graphic reference made of an array of interconnected tiles. The square tile is aligned with the XY plane, and the block provides frame connector ports to the middle points on each of the four sides of the body of the square - right (+X), left (-X), top (+Y) and bottom (-Y). All dimensions are in meters.
      settings: PortSchema="{\"entries\":[{\"content\":{\"sides\":[{\"content\":{\"connectorIds\":[\"LConn1\"]},\"type\":\"ConnectorPlacement.EquallySpacedRectSide\",\"uuid\":\"a971723f-ea37-4e9b-910b-501b94fb0ba2\"},{\"content\":{\"connectorIds\":[\"RConn1\"],\"side\":\"RIGHT\"},\"type\":\"ConnectorPlacement.EquallySpacedRectSide\",\"uuid\":\"e50175c1-005c-4b0b-bced-b882197eaab2\"},{\"content\":{\"connectorIds\":[\"LConn2\"],\"side\":\"TOP\"},\"type\":\"ConnectorPlacement.EquallySpacedRectSide\",\"uuid\":\"2a04a964-d53e-47ee-8c79-d53dd599bafe\"},{\"content\":{\"connectorIds\":[\"RConn2\"],\"side\":\"BOTTOM\"},\"type\":\"ConnectorPlacement.EquallySpacedRectSide\",\"uuid\":\"a0066dd6-a193-491c-afbe-bac00dfc3505\"}]},\"type\":\"ConnectorPlacement.EquallySpacedConnector\",\"uuid\":\"c80211c6-bb24-481b-97ca-2752015f3b18\"}],\"packageUris\":[\"http://schema.mathworks.com/mf0/Connector/19700101\"],\"version\":\"1.0\"}"
  Tile82 : Subsystem  mask(Square Tile){side=side, thickness=thick, color=color2, opacity=opacity}
